simulink model "K_Sim_NoCap"  (R2020b)
settings: Solver=FixedStepAuto  StartTime=0  StopTime=2  FixedStep=Ts  RelTol=1e-3
undefined symbols (not defined in the file or in its folder): DeviceDiscreDamping, DevicePara, DevicePowerFlow, DeviceType, Fbase, OtherInputs, Sbase, Ts, Vbase, Wbase, x_e, Zbase
libraries: powerlib x155, SimplexPS x119
(part 1 of 2)
settings Model: Creator=admin_user  LastModifiedBy=admin_user

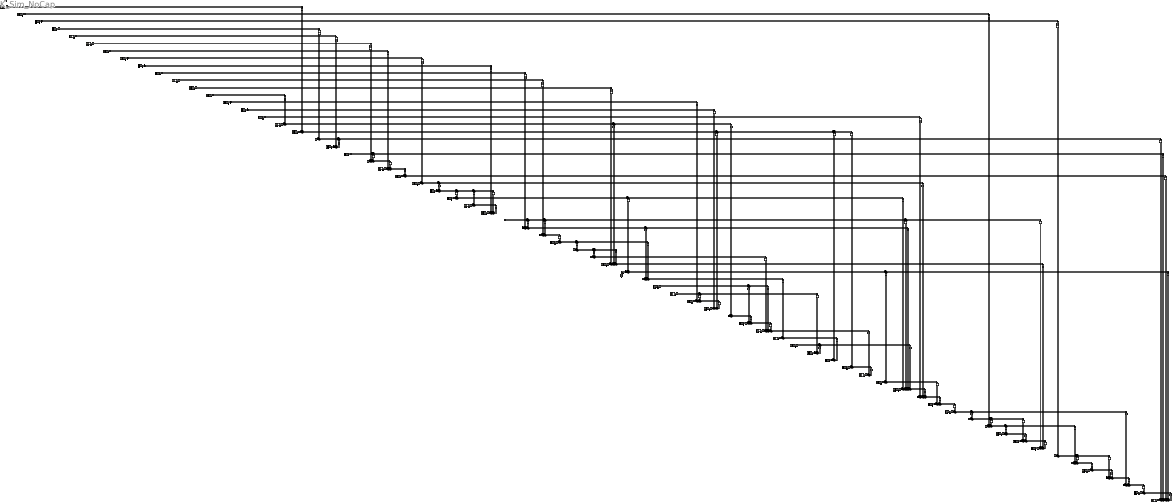
== system K_Sim_NoCap ==
  Branch1-18 : powerlib/Elements/Three-Phase Series RLC Branch  LConnTagsString=A|B|C  RConnTagsString=A|B|C  BranchType=RL  Resistance=(1e-07)*Zbase  Inductance=(0.003)*Zbase/Wbase  Capacitance=1e-6  Measurements=None
  Branch10-31 : powerlib/Elements/Three-Phase Series RLC Branch  LConnTagsString=A|B|C  RConnTagsString=A|B|C  BranchType=RL  Resistance=(1e-07)*Zbase  Inductance=(0.026)*Zbase/Wbase  Capacitance=1e-6  Measurements=None
  Branch11-32 : powerlib/Elements/Three-Phase Series RLC Branch  LConnTagsString=A|B|C  RConnTagsString=A|B|C  BranchType=RL  Resistance=(1e-07)*Zbase  Inductance=(0.013)*Zbase/Wbase  Capacitance=1e-6  Measurements=None
  Branch12-36 : powerlib/Elements/Three-Phase Series RLC Branch  LConnTagsString=A|B|C  RConnTagsString=A|B|C  BranchType=RL  Resistance=(1e-07)*Zbase  Inductance=(0.0075)*Zbase/Wbase  Capacitance=1e-6  Measurements=None
  Branch13-17 : powerlib/Elements/Three-Phase Series RLC Branch  LConnTagsString=A|B|C  RConnTagsString=A|B|C  BranchType=RL  Resistance=(1e-07)*Zbase  Inductance=(0.0033)*Zbase/Wbase  Capacitance=1e-6  Measurements=None
  Branch14-41 : powerlib/Elements/Three-Phase Series RLC Branch  LConnTagsString=A|B|C  RConnTagsString=A|B|C  BranchType=RL  Resistance=(1e-07)*Zbase  Inductance=(0.0015)*Zbase/Wbase  Capacitance=1e-6  Measurements=None
  Branch15-42 : powerlib/Elements/Three-Phase Series RLC Branch  LConnTagsString=A|B|C  RConnTagsString=A|B|C  BranchType=RL  Resistance=(1e-07)*Zbase  Inductance=(0.0015)*Zbase/Wbase  Capacitance=1e-6  Measurements=None
  Branch16-54 : powerlib/Elements/Three-Phase Series RLC Branch  LConnTagsString=A|B|C  RConnTagsString=A|B|C  BranchType=RL  Resistance=(1e-07)*Zbase  Inductance=(0.0181)*Zbase/Wbase  Capacitance=1e-6  Measurements=None
  Branch17-36 : powerlib/Elements/Three-Phase Series RLC Branch  LConnTagsString=A|B|C  RConnTagsString=A|B|C  BranchType=RL  Resistance=(0.0005)*Zbase  Inductance=(0.0045)*Zbase/Wbase  Capacitance=1e-6  Measurements=None
  Branch17-43 : powerlib/Elements/Three-Phase Series RLC Branch  LConnTagsString=A|B|C  RConnTagsString=A|B|C  BranchType=RL  Resistance=(0.0005)*Zbase  Inductance=(0.0276)*Zbase/Wbase  Capacitance=1e-6  Measurements=None
  Branch18-42 : powerlib/Elements/Three-Phase Series RLC Branch  LConnTagsString=A|B|C  RConnTagsString=A|B|C  BranchType=RL  Resistance=(0.004)*Zbase  Inductance=(0.06)*Zbase/Wbase  Capacitance=1e-6  Measurements=None
  Branch18-49 : powerlib/Elements/Three-Phase Series RLC Branch  LConnTagsString=A|B|C  RConnTagsString=A|B|C  BranchType=RL  Resistance=(0.0076)*Zbase  Inductance=(0.1141)*Zbase/Wbase  Capacitance=1e-6  Measurements=None
  Branch18-50 : powerlib/Elements/Three-Phase Series RLC Branch  LConnTagsString=A|B|C  RConnTagsString=A|B|C  BranchType=RL  Resistance=(0.0012)*Zbase  Inductance=(0.0288)*Zbase/Wbase  Capacitance=1e-6  Measurements=None
  Branch19-20 : powerlib/Elements/Three-Phase Series RLC Branch  LConnTagsString=A|B|C  RConnTagsString=A|B|C  BranchType=RL  Resistance=(0.00078652)*Zbase  Inductance=(0.015506)*Zbase/Wbase  Capacitance=1e-6  Measurements=None
  Branch19-68 : powerlib/Elements/Three-Phase Series RLC Branch  LConnTagsString=A|B|C  RConnTagsString=A|B|C  BranchType=RL  Resistance=(0.0016)*Zbase  Inductance=(0.0195)*Zbase/Wbase  Capacitance=1e-6  Measurements=None
  Branch2-58 : powerlib/Elements/Three-Phase Series RLC Branch  LConnTagsString=A|B|C  RConnTagsString=A|B|C  BranchType=RL  Resistance=(1e-07)*Zbase  Inductance=(0.025)*Zbase/Wbase  Capacitance=1e-6  Measurements=None
  Branch21-22 : powerlib/Elements/Three-Phase Series RLC Branch  LConnTagsString=A|B|C  RConnTagsString=A|B|C  BranchType=RL  Resistance=(0.0008)*Zbase  Inductance=(0.014)*Zbase/Wbase  Capacitance=1e-6  Measurements=None
  Branch21-68 : powerlib/Elements/Three-Phase Series RLC Branch  LConnTagsString=A|B|C  RConnTagsString=A|B|C  BranchType=RL  Resistance=(0.0008)*Zbase  Inductance=(0.0135)*Zbase/Wbase  Capacitance=1e-6  Measurements=None
  Branch22-23 : powerlib/Elements/Three-Phase Series RLC Branch  LConnTagsString=A|B|C  RConnTagsString=A|B|C  BranchType=RL  Resistance=(0.0006)*Zbase  Inductance=(0.0096)*Zbase/Wbase  Capacitance=1e-6  Measurements=None
  Branch23-24 : powerlib/Elements/Three-Phase Series RLC Branch  LConnTagsString=A|B|C  RConnTagsString=A|B|C  BranchType=RL  Resistance=(0.0022)*Zbase  Inductance=(0.035)*Zbase/Wbase  Capacitance=1e-6  Measurements=None
  Branch24-68 : powerlib/Elements/Three-Phase Series RLC Branch  LConnTagsString=A|B|C  RConnTagsString=A|B|C  BranchType=RL  Resistance=(0.0003)*Zbase  Inductance=(0.0059)*Zbase/Wbase  Capacitance=1e-6  Measurements=None
  Branch25-26 : powerlib/Elements/Three-Phase Series RLC Branch  LConnTagsString=A|B|C  RConnTagsString=A|B|C  BranchType=RL  Resistance=(0.0032)*Zbase  Inductance=(0.0323)*Zbase/Wbase  Capacitance=1e-6  Measurements=None
  Branch25-54 : powerlib/Elements/Three-Phase Series RLC Branch  LConnTagsString=A|B|C  RConnTagsString=A|B|C  BranchType=RL  Resistance=(0.007)*Zbase  Inductance=(0.0086)*Zbase/Wbase  Capacitance=1e-6  Measurements=None
  Branch26-27 : powerlib/Elements/Three-Phase Series RLC Branch  LConnTagsString=A|B|C  RConnTagsString=A|B|C  BranchType=RL  Resistance=(0.0014)*Zbase  Inductance=(0.0147)*Zbase/Wbase  Capacitance=1e-6  Measurements=None
  Branch26-28 : powerlib/Elements/Three-Phase Series RLC Branch  LConnTagsString=A|B|C  RConnTagsString=A|B|C  BranchType=RL  Resistance=(0.0043)*Zbase  Inductance=(0.0474)*Zbase/Wbase  Capacitance=1e-6  Measurements=None
  Branch26-29 : powerlib/Elements/Three-Phase Series RLC Branch  LConnTagsString=A|B|C  RConnTagsString=A|B|C  BranchType=RL  Resistance=(0.0057)*Zbase  Inductance=(0.0625)*Zbase/Wbase  Capacitance=1e-6  Measurements=None
  Branch27-37 : powerlib/Elements/Three-Phase Series RLC Branch  LConnTagsString=A|B|C  RConnTagsString=A|B|C  BranchType=RL  Resistance=(0.0013)*Zbase  Inductance=(0.0173)*Zbase/Wbase  Capacitance=1e-6  Measurements=None
  Branch27-53 : powerlib/Elements/Three-Phase Series RLC Branch  LConnTagsString=A|B|C  RConnTagsString=A|B|C  BranchType=RL  Resistance=(0.032)*Zbase  Inductance=(0.32)*Zbase/Wbase  Capacitance=1e-6  Measurements=None
  Branch28-29 : powerlib/Elements/Three-Phase Series RLC Branch  LConnTagsString=A|B|C  RConnTagsString=A|B|C  BranchType=RL  Resistance=(0.0014)*Zbase  Inductance=(0.0151)*Zbase/Wbase  Capacitance=1e-6  Measurements=None
  Branch3-62 : powerlib/Elements/Three-Phase Series RLC Branch  LConnTagsString=A|B|C  RConnTagsString=A|B|C  BranchType=RL  Resistance=(1e-07)*Zbase  Inductance=(0.02)*Zbase/Wbase  Capacitance=1e-6  Measurements=None
  Branch30-31 : powerlib/Elements/Three-Phase Series RLC Branch  LConnTagsString=A|B|C  RConnTagsString=A|B|C  BranchType=RL  Resistance=(0.0013)*Zbase  Inductance=(0.0187)*Zbase/Wbase  Capacitance=1e-6  Measurements=None
  Branch30-32 : powerlib/Elements/Three-Phase Series RLC Branch  LConnTagsString=A|B|C  RConnTagsString=A|B|C  BranchType=RL  Resistance=(0.0024)*Zbase  Inductance=(0.0288)*Zbase/Wbase  Capacitance=1e-6  Measurements=None
  Branch30-53 : powerlib/Elements/Three-Phase Series RLC Branch  LConnTagsString=A|B|C  RConnTagsString=A|B|C  BranchType=RL  Resistance=(0.0008)*Zbase  Inductance=(0.0074)*Zbase/Wbase  Capacitance=1e-6  Measurements=None
  Branch30-61 : powerlib/Elements/Three-Phase Series RLC Branch  LConnTagsString=A|B|C  RConnTagsString=A|B|C  BranchType=RL  Resistance=(0.00095)*Zbase  Inductance=(0.00915)*Zbase/Wbase  Capacitance=1e-6  Measurements=None
  Branch31-38 : powerlib/Elements/Three-Phase Series RLC Branch  LConnTagsString=A|B|C  RConnTagsString=A|B|C  BranchType=RL  Resistance=(0.0011)*Zbase  Inductance=(0.0147)*Zbase/Wbase  Capacitance=1e-6  Measurements=None
  Branch31-53 : powerlib/Elements/Three-Phase Series RLC Branch  LConnTagsString=A|B|C  RConnTagsString=A|B|C  BranchType=RL  Resistance=(0.0016)*Zbase  Inductance=(0.0163)*Zbase/Wbase  Capacitance=1e-6  Measurements=None
  Branch32-33 : powerlib/Elements/Three-Phase Series RLC Branch  LConnTagsString=A|B|C  RConnTagsString=A|B|C  BranchType=RL  Resistance=(0.0008)*Zbase  Inductance=(0.0099)*Zbase/Wbase  Capacitance=1e-6  Measurements=None
  Branch33-34 : powerlib/Elements/Three-Phase Series RLC Branch  LConnTagsString=A|B|C  RConnTagsString=A|B|C  BranchType=RL  Resistance=(0.0011)*Zbase  Inductance=(0.0157)*Zbase/Wbase  Capacitance=1e-6  Measurements=None
  Branch33-38 : powerlib/Elements/Three-Phase Series RLC Branch  LConnTagsString=A|B|C  RConnTagsString=A|B|C  BranchType=RL  Resistance=(0.0036)*Zbase  Inductance=(0.0444)*Zbase/Wbase  Capacitance=1e-6  Measurements=None
  Branch34-35 : powerlib/Elements/Three-Phase Series RLC Branch  LConnTagsString=A|B|C  RConnTagsString=A|B|C  BranchType=RL  Resistance=(0.0001)*Zbase  Inductance=(0.0074)*Zbase/Wbase  Capacitance=1e-6  Measurements=None
  Branch34-36 : powerlib/Elements/Three-Phase Series RLC Branch  LConnTagsString=A|B|C  RConnTagsString=A|B|C  BranchType=RL  Resistance=(0.0033)*Zbase  Inductance=(0.0111)*Zbase/Wbase  Capacitance=1e-6  Measurements=None
  Branch35-45 : powerlib/Elements/Three-Phase Series RLC Branch  LConnTagsString=A|B|C  RConnTagsString=A|B|C  BranchType=RL  Resistance=(0.0007)*Zbase  Inductance=(0.0175)*Zbase/Wbase  Capacitance=1e-6  Measurements=None
  Branch36-61 : powerlib/Elements/Three-Phase Series RLC Branch  LConnTagsString=A|B|C  RConnTagsString=A|B|C  BranchType=RL  Resistance=(0.0011)*Zbase  Inductance=(0.0098)*Zbase/Wbase  Capacitance=1e-6  Measurements=None
  Branch37-52 : powerlib/Elements/Three-Phase Series RLC Branch  LConnTagsString=A|B|C  RConnTagsString=A|B|C  BranchType=RL  Resistance=(0.0007)*Zbase  Inductance=(0.0082)*Zbase/Wbase  Capacitance=1e-6  Measurements=None
  Branch37-68 : powerlib/Elements/Three-Phase Series RLC Branch  LConnTagsString=A|B|C  RConnTagsString=A|B|C  BranchType=RL  Resistance=(0.0007)*Zbase  Inductance=(0.0089)*Zbase/Wbase  Capacitance=1e-6  Measurements=None
  Branch38-46 : powerlib/Elements/Three-Phase Series RLC Branch  LConnTagsString=A|B|C  RConnTagsString=A|B|C  BranchType=RL  Resistance=(0.0022)*Zbase  Inductance=(0.0284)*Zbase/Wbase  Capacitance=1e-6  Measurements=None
  Branch39-44 : powerlib/Elements/Three-Phase Series RLC Branch  LConnTagsString=A|B|C  RConnTagsString=A|B|C  BranchType=RL  Resistance=(1e-07)*Zbase  Inductance=(0.0411)*Zbase/Wbase  Capacitance=1e-6  Measurements=None
  Branch39-45 : powerlib/Elements/Three-Phase Series RLC Branch  LConnTagsString=A|B|C  RConnTagsString=A|B|C  BranchType=RL  Resistance=(1e-07)*Zbase  Inductance=(0.0839)*Zbase/Wbase  Capacitance=1e-6  Measurements=None
  Branch4-19 : powerlib/Elements/Three-Phase Series RLC Branch  LConnTagsString=A|B|C  RConnTagsString=A|B|C  BranchType=RL  Resistance=(0.0007)*Zbase  Inductance=(0.0142)*Zbase/Wbase  Capacitance=1e-6  Measurements=None
  Branch40-41 : powerlib/Elements/Three-Phase Series RLC Branch  LConnTagsString=A|B|C  RConnTagsString=A|B|C  BranchType=RL  Resistance=(0.006)*Zbase  Inductance=(0.084)*Zbase/Wbase  Capacitance=1e-6  Measurements=None
  Branch40-48 : powerlib/Elements/Three-Phase Series RLC Branch  LConnTagsString=A|B|C  RConnTagsString=A|B|C  BranchType=RL  Resistance=(0.002)*Zbase  Inductance=(0.022)*Zbase/Wbase  Capacitance=1e-6  Measurements=None
  Branch41-42 : powerlib/Elements/Three-Phase Series RLC Branch  LConnTagsString=A|B|C  RConnTagsString=A|B|C  BranchType=RL  Resistance=(0.004)*Zbase  Inductance=(0.06)*Zbase/Wbase  Capacitance=1e-6  Measurements=None
  Branch43-44 : powerlib/Elements/Three-Phase Series RLC Branch  LConnTagsString=A|B|C  RConnTagsString=A|B|C  BranchType=RL  Resistance=(0.0001)*Zbase  Inductance=(0.0011)*Zbase/Wbase  Capacitance=1e-6  Measurements=None
  Branch44-45 : powerlib/Elements/Three-Phase Series RLC Branch  LConnTagsString=A|B|C  RConnTagsString=A|B|C  BranchType=RL  Resistance=(0.0025)*Zbase  Inductance=(0.073)*Zbase/Wbase  Capacitance=1e-6  Measurements=None
  Branch45-51 : powerlib/Elements/Three-Phase Series RLC Branch  LConnTagsString=A|B|C  RConnTagsString=A|B|C  BranchType=RL  Resistance=(0.0004)*Zbase  Inductance=(0.0105)*Zbase/Wbase  Capacitance=1e-6  Measurements=None
  Branch46-49 : powerlib/Elements/Three-Phase Series RLC Branch  LConnTagsString=A|B|C  RConnTagsString=A|B|C  BranchType=RL  Resistance=(0.0018)*Zbase  Inductance=(0.0274)*Zbase/Wbase  Capacitance=1e-6  Measurements=None
  Branch47-48 : powerlib/Elements/Three-Phase Series RLC Branch  LConnTagsString=A|B|C  RConnTagsString=A|B|C  BranchType=RL  Resistance=(0.00125)*Zbase  Inductance=(0.0134)*Zbase/Wbase  Capacitance=1e-6  Measurements=None
  Branch47-53 : powerlib/Elements/Three-Phase Series RLC Branch  LConnTagsString=A|B|C  RConnTagsString=A|B|C  BranchType=RL  Resistance=(0.0013)*Zbase  Inductance=(0.0188)*Zbase/Wbase  Capacitance=1e-6  Measurements=None
  Branch5-20 : powerlib/Elements/Three-Phase Series RLC Branch  LConnTagsString=A|B|C  RConnTagsString=A|B|C  BranchType=RL  Resistance=(0.0009)*Zbase  Inductance=(0.018)*Zbase/Wbase  Capacitance=1e-6  Measurements=None
  Branch50-51 : powerlib/Elements/Three-Phase Series RLC Branch  LConnTagsString=A|B|C  RConnTagsString=A|B|C  BranchType=RL  Resistance=(0.0009)*Zbase  Inductance=(0.0221)*Zbase/Wbase  Capacitance=1e-6  Measurements=None
  Branch52-55 : powerlib/Elements/Three-Phase Series RLC Branch  LConnTagsString=A|B|C  RConnTagsString=A|B|C  BranchType=RL  Resistance=(0.0011)*Zbase  Inductance=(0.0133)*Zbase/Wbase  Capacitance=1e-6  Measurements=None
  Branch53-54 : powerlib/Elements/Three-Phase Series RLC Branch  LConnTagsString=A|B|C  RConnTagsString=A|B|C  BranchType=RL  Resistance=(0.0035)*Zbase  Inductance=(0.0411)*Zbase/Wbase  Capacitance=1e-6  Measurements=None
  Branch54-55 : powerlib/Elements/Three-Phase Series RLC Branch  LConnTagsString=A|B|C  RConnTagsString=A|B|C  BranchType=RL  Resistance=(0.0013)*Zbase  Inductance=(0.0151)*Zbase/Wbase  Capacitance=1e-6  Measurements=None
  Branch55-56 : powerlib/Elements/Three-Phase Series RLC Branch  LConnTagsString=A|B|C  RConnTagsString=A|B|C  BranchType=RL  Resistance=(0.0013)*Zbase  Inductance=(0.0213)*Zbase/Wbase  Capacitance=1e-6  Measurements=None
  Branch56-57 : powerlib/Elements/Three-Phase Series RLC Branch  LConnTagsString=A|B|C  RConnTagsString=A|B|C  BranchType=RL  Resistance=(0.0008)*Zbase  Inductance=(0.0128)*Zbase/Wbase  Capacitance=1e-6  Measurements=None
  Branch56-66 : powerlib/Elements/Three-Phase Series RLC Branch  LConnTagsString=A|B|C  RConnTagsString=A|B|C  BranchType=RL  Resistance=(0.0008)*Zbase  Inductance=(0.0129)*Zbase/Wbase  Capacitance=1e-6  Measurements=None
  Branch57-58 : powerlib/Elements/Three-Phase Series RLC Branch  LConnTagsString=A|B|C  RConnTagsString=A|B|C  BranchType=RL  Resistance=(0.0002)*Zbase  Inductance=(0.0026)*Zbase/Wbase  Capacitance=1e-6  Measurements=None
  Branch57-60 : powerlib/Elements/Three-Phase Series RLC Branch  LConnTagsString=A|B|C  RConnTagsString=A|B|C  BranchType=RL  Resistance=(0.0008)*Zbase  Inductance=(0.0112)*Zbase/Wbase  Capacitance=1e-6  Measurements=None
  Branch58-59 : powerlib/Elements/Three-Phase Series RLC Branch  LConnTagsString=A|B|C  RConnTagsString=A|B|C  BranchType=RL  Resistance=(0.0006)*Zbase  Inductance=(0.0092)*Zbase/Wbase  Capacitance=1e-6  Measurements=None
  Branch58-63 : powerlib/Elements/Three-Phase Series RLC Branch  LConnTagsString=A|B|C  RConnTagsString=A|B|C  BranchType=RL  Resistance=(0.0007)*Zbase  Inductance=(0.0082)*Zbase/Wbase  Capacitance=1e-6  Measurements=None
  Branch59-60 : powerlib/Elements/Three-Phase Series RLC Branch  LConnTagsString=A|B|C  RConnTagsString=A|B|C  BranchType=RL  Resistance=(0.0004)*Zbase  Inductance=(0.0046)*Zbase/Wbase  Capacitance=1e-6  Measurements=None
  Branch6-22 : powerlib/Elements/Three-Phase Series RLC Branch  LConnTagsString=A|B|C  RConnTagsString=A|B|C  BranchType=RL  Resistance=(1e-07)*Zbase  Inductance=(0.0143)*Zbase/Wbase  Capacitance=1e-6  Measurements=None
  Branch60-61 : powerlib/Elements/Three-Phase Series RLC Branch  LConnTagsString=A|B|C  RConnTagsString=A|B|C  BranchType=RL  Resistance=(0.0023)*Zbase  Inductance=(0.0363)*Zbase/Wbase  Capacitance=1e-6  Measurements=None
  Branch62-63 : powerlib/Elements/Three-Phase Series RLC Branch  LConnTagsString=A|B|C  RConnTagsString=A|B|C  BranchType=RL  Resistance=(0.0004)*Zbase  Inductance=(0.0043)*Zbase/Wbase  Capacitance=1e-6  Measurements=None
  Branch62-65 : powerlib/Elements/Three-Phase Series RLC Branch  LConnTagsString=A|B|C  RConnTagsString=A|B|C  BranchType=RL  Resistance=(0.0004)*Zbase  Inductance=(0.0043)*Zbase/Wbase  Capacitance=1e-6  Measurements=None
  Branch63-64 : powerlib/Elements/Three-Phase Series RLC Branch  LConnTagsString=A|B|C  RConnTagsString=A|B|C  BranchType=RL  Resistance=(0.0016)*Zbase  Inductance=(0.0435)*Zbase/Wbase  Capacitance=1e-6  Measurements=None
  Branch64-65 : powerlib/Elements/Three-Phase Series RLC Branch  LConnTagsString=A|B|C  RConnTagsString=A|B|C  BranchType=RL  Resistance=(0.0017978)*Zbase  Inductance=(0.048877)*Zbase/Wbase  Capacitance=1e-6  Measurements=None
  Branch65-66 : powerlib/Elements/Three-Phase Series RLC Branch  LConnTagsString=A|B|C  RConnTagsString=A|B|C  BranchType=RL  Resistance=(0.0009)*Zbase  Inductance=(0.0101)*Zbase/Wbase  Capacitance=1e-6  Measurements=None
  Branch66-67 : powerlib/Elements/Three-Phase Series RLC Branch  LConnTagsString=A|B|C  RConnTagsString=A|B|C  BranchType=RL  Resistance=(0.0018)*Zbase  Inductance=(0.0217)*Zbase/Wbase  Capacitance=1e-6  Measurements=None
  Branch67-68 : powerlib/Elements/Three-Phase Series RLC Branch  LConnTagsString=A|B|C  RConnTagsString=A|B|C  BranchType=RL  Resistance=(0.0009)*Zbase  Inductance=(0.0094)*Zbase/Wbase  Capacitance=1e-6  Measurements=None
  Branch7-23 : powerlib/Elements/Three-Phase Series RLC Branch  LConnTagsString=A|B|C  RConnTagsString=A|B|C  BranchType=RL  Resistance=(0.0005)*Zbase  Inductance=(0.0272)*Zbase/Wbase  Capacitance=1e-6  Measurements=None
  Branch8-25 : powerlib/Elements/Three-Phase Series RLC Branch  LConnTagsString=A|B|C  RConnTagsString=A|B|C  BranchType=RL  Resistance=(0.0006)*Zbase  Inductance=(0.0232)*Zbase/Wbase  Capacitance=1e-6  Measurements=None
  Branch9-29 : powerlib/Elements/Three-Phase Series RLC Branch  LConnTagsString=A|B|C  RConnTagsString=A|B|C  BranchType=RL  Resistance=(0.0008)*Zbase  Inductance=(0.0156)*Zbase/Wbase  Capacitance=1e-6  Measurements=None
  Bus{1..68} (68 alike) : SimplexPS/Three-Phase Bus  Vbase=1  Sbase=1
      settings: SourceProductName=Simplex Power Systems
  Current Measurement1 : powerlib/Measurements/Current Measurement  PhasorSimulation=off  OutputType=Complex  PSBequivalent=0
  D-GND{1..18,20..29,33,36,39..42,44..53,55..56,59..61,64,67..68} (52 alike) : powerlib/Elements/Ground  LConnTagsString=a
  D-Scope{1..18,20..21,23..29,33,36,39..42,44..53,55..56,59..61,64,67..68} (51 alike) : Scope  NumInputPorts=7
  DS-Bus{1..18,20..21,23..29,33,36,39..42,44..53,55..56,59..61,64,67..68} (51 alike) : BusSelector  OutputSignals=v_dq,i_dq,v_abc,i_abc,w,theta,pq
  Load Impulse1 : Subsystem  AncestorBlock=SimplexPS/Load Impulse  mask{t0=1, dt=3/60, R=1e-9*Zbase}
  Scope1 : Scope
  Transformer10-31 : powerlib/Elements/Three-Phase Transformer (Two Windings)  Winding1Connection=Yg  Winding2Connection=Yg  CoreType=Three single-phase transformers  SetSaturation=off  Hysteresis=off  DataFile='hysteresis'  SetInitialFlux=off  Measurements=None  UNITS=pu  NominalPower=[Sbase, Fbase]  Winding1=[1.04*Vbase, 0, 0]  Winding2=[Vbase, 0, 0]  Rm=1e4  Lm=1e4  L0=0.5  Saturation=[ 0,0 ; 0.0024,1.2 ; 1.0,1.52 ]  InitialFluxes=[ 0.8 , -0.8 , 0.7 ]  BreakLoop=off  DiscreteSolver=Trapezoidal iterative  DataType=off  TransfoNumber=1
  Transformer11-32 : powerlib/Elements/Three-Phase Transformer (Two Windings)  Winding1Connection=Yg  Winding2Connection=Yg  CoreType=Three single-phase transformers  SetSaturation=off  Hysteresis=off  DataFile='hysteresis'  SetInitialFlux=off  Measurements=None  UNITS=pu  NominalPower=[Sbase, Fbase]  Winding1=[1.04*Vbase, 0, 0]  Winding2=[Vbase, 0, 0]  Rm=1e4  Lm=1e4  L0=0.5  Saturation=[ 0,0 ; 0.0024,1.2 ; 1.0,1.52 ]  InitialFluxes=[ 0.8 , -0.8 , 0.7 ]  BreakLoop=off  DiscreteSolver=Trapezoidal iterative  DataType=off  TransfoNumber=1
  Transformer12-36 : powerlib/Elements/Three-Phase Transformer (Two Windings)  Winding1Connection=Yg  Winding2Connection=Yg  CoreType=Three single-phase transformers  SetSaturation=off  Hysteresis=off  DataFile='hysteresis'  SetInitialFlux=off  Measurements=None  UNITS=pu  NominalPower=[Sbase, Fbase]  Winding1=[1.04*Vbase, 0, 0]  Winding2=[Vbase, 0, 0]  Rm=1e4  Lm=1e4  L0=0.5  Saturation=[ 0,0 ; 0.0024,1.2 ; 1.0,1.52 ]  InitialFluxes=[ 0.8 , -0.8 , 0.7 ]  BreakLoop=off  DiscreteSolver=Trapezoidal iterative  DataType=off  TransfoNumber=1
  Transformer13-17 : powerlib/Elements/Three-Phase Transformer (Two Windings)  Winding1Connection=Yg  Winding2Connection=Yg  CoreType=Three single-phase transformers  SetSaturation=off  Hysteresis=off  DataFile='hysteresis'  SetInitialFlux=off  Measurements=None  UNITS=pu  NominalPower=[Sbase, Fbase]  Winding1=[1.04*Vbase, 0, 0]  Winding2=[Vbase, 0, 0]  Rm=1e4  Lm=1e4  L0=0.5  Saturation=[ 0,0 ; 0.0024,1.2 ; 1.0,1.52 ]  InitialFluxes=[ 0.8 , -0.8 , 0.7 ]  BreakLoop=off  DiscreteSolver=Trapezoidal iterative  DataType=off  TransfoNumber=1
  Transformer16-54 : powerlib/Elements/Three-Phase Transformer (Two Windings)  Winding1Connection=Yg  Winding2Connection=Yg  CoreType=Three single-phase transformers  SetSaturation=off  Hysteresis=off  DataFile='hysteresis'  SetInitialFlux=off  Measurements=None  UNITS=pu  NominalPower=[Sbase, Fbase]  Winding1=[1.025*Vbase, 0, 0]  Winding2=[Vbase, 0, 0]  Rm=1e4  Lm=1e4  L0=0.5  Saturation=[ 0,0 ; 0.0024,1.2 ; 1.0,1.52 ]  InitialFluxes=[ 0.8 , -0.8 , 0.7 ]  BreakLoop=off  DiscreteSolver=Trapezoidal iterative  DataType=off  TransfoNumber=1
  Transformer19-20 : powerlib/Elements/Three-Phase Transformer (Two Windings)  Winding1Connection=Yg  Winding2Connection=Yg  CoreType=Three single-phase transformers  SetSaturation=off  Hysteresis=off  DataFile='hysteresis'  SetInitialFlux=off  Measurements=None  UNITS=pu  NominalPower=[Sbase, Fbase]  Winding1=[0.9434*Vbase, 0, 0]  Winding2=[Vbase, 0, 0]  Rm=1e4  Lm=1e4  L0=0.5  Saturation=[ 0,0 ; 0.0024,1.2 ; 1.0,1.52 ]  InitialFluxes=[ 0.8 , -0.8 , 0.7 ]  BreakLoop=off  DiscreteSolver=Trapezoidal iterative  DataType=off  TransfoNumber=1
  Transformer2-58 : powerlib/Elements/Three-Phase Transformer (Two Windings)  Winding1Connection=Yg  Winding2Connection=Yg  CoreType=Three single-phase transformers  SetSaturation=off  Hysteresis=off  DataFile='hysteresis'  SetInitialFlux=off  Measurements=None  UNITS=pu  NominalPower=[Sbase, Fbase]  Winding1=[1.07*Vbase, 0, 0]  Winding2=[Vbase, 0, 0]  Rm=1e4  Lm=1e4  L0=0.5  Saturation=[ 0,0 ; 0.0024,1.2 ; 1.0,1.52 ]  InitialFluxes=[ 0.8 , -0.8 , 0.7 ]  BreakLoop=off  DiscreteSolver=Trapezoidal iterative  DataType=off  TransfoNumber=1
  Transformer3-62 : powerlib/Elements/Three-Phase Transformer (Two Windings)  Winding1Connection=Yg  Winding2Connection=Yg  CoreType=Three single-phase transformers  SetSaturation=off  Hysteresis=off  DataFile='hysteresis'  SetInitialFlux=off  Measurements=None  UNITS=pu  NominalPower=[Sbase, Fbase]  Winding1=[1.07*Vbase, 0, 0]  Winding2=[Vbase, 0, 0]  Rm=1e4  Lm=1e4  L0=0.5  Saturation=[ 0,0 ; 0.0024,1.2 ; 1.0,1.52 ]  InitialFluxes=[ 0.8 , -0.8 , 0.7 ]  BreakLoop=off  DiscreteSolver=Trapezoidal iterative  DataType=off  TransfoNumber=1
  Transformer34-35 : powerlib/Elements/Three-Phase Transformer (Two Windings)  Winding1Connection=Yg  Winding2Connection=Yg  CoreType=Three single-phase transformers  SetSaturation=off  Hysteresis=off  DataFile='hysteresis'  SetInitialFlux=off  Measurements=None  UNITS=pu  NominalPower=[Sbase, Fbase]  Winding1=[0.946*Vbase, 0, 0]  Winding2=[Vbase, 0, 0]  Rm=1e4  Lm=1e4  L0=0.5  Saturation=[ 0,0 ; 0.0024,1.2 ; 1.0,1.52 ]  InitialFluxes=[ 0.8 , -0.8 , 0.7 ]  BreakLoop=off  DiscreteSolver=Trapezoidal iterative  DataType=off  TransfoNumber=1
  Transformer4-19 : powerlib/Elements/Three-Phase Transformer (Two Windings)  Winding1Connection=Yg  Winding2Connection=Yg  CoreType=Three single-phase transformers  SetSaturation=off  Hysteresis=off  DataFile='hysteresis'  SetInitialFlux=off  Measurements=None  UNITS=pu  NominalPower=[Sbase, Fbase]  Winding1=[1.07*Vbase, 0, 0]  Winding2=[Vbase, 0, 0]  Rm=1e4  Lm=1e4  L0=0.5  Saturation=[ 0,0 ; 0.0024,1.2 ; 1.0,1.52 ]  InitialFluxes=[ 0.8 , -0.8 , 0.7 ]  BreakLoop=off  DiscreteSolver=Trapezoidal iterative  DataType=off  TransfoNumber=1
  Transformer5-20 : powerlib/Elements/Three-Phase Transformer (Two Windings)  Winding1Connection=Yg  Winding2Connection=Yg  CoreType=Three single-phase transformers  SetSaturation=off  Hysteresis=off  DataFile='hysteresis'  SetInitialFlux=off  Measurements=None  UNITS=pu  NominalPower=[Sbase, Fbase]  Winding1=[1.009*Vbase, 0, 0]  Winding2=[Vbase, 0, 0]  Rm=1e4  Lm=1e4  L0=0.5  Saturation=[ 0,0 ; 0.0024,1.2 ; 1.0,1.52 ]  InitialFluxes=[ 0.8 , -0.8 , 0.7 ]  BreakLoop=off  DiscreteSolver=Trapezoidal iterative  DataType=off  TransfoNumber=1
  Transformer6-22 : powerlib/Elements/Three-Phase Transformer (Two Windings)  Winding1Connection=Yg  Winding2Connection=Yg  CoreType=Three single-phase transformers  SetSaturation=off  Hysteresis=off  DataFile='hysteresis'  SetInitialFlux=off  Measurements=None  UNITS=pu  NominalPower=[Sbase, Fbase]  Winding1=[1.025*Vbase, 0, 0]  Winding2=[Vbase, 0, 0]  Rm=1e4  Lm=1e4  L0=0.5  Saturation=[ 0,0 ; 0.0024,1.2 ; 1.0,1.52 ]  InitialFluxes=[ 0.8 , -0.8 , 0.7 ]  BreakLoop=off  DiscreteSolver=Trapezoidal iterative  DataType=off  TransfoNumber=1
  Transformer63-64 : powerlib/Elements/Three-Phase Transformer (Two Windings)  Winding1Connection=Yg  Winding2Connection=Yg  CoreType=Three single-phase transformers  SetSaturation=off  Hysteresis=off  DataFile='hysteresis'  SetInitialFlux=off  Measurements=None  UNITS=pu  NominalPower=[Sbase, Fbase]  Winding1=[1.06*Vbase, 0, 0]  Winding2=[Vbase, 0, 0]  Rm=1e4  Lm=1e4  L0=0.5  Saturation=[ 0,0 ; 0.0024,1.2 ; 1.0,1.52 ]  InitialFluxes=[ 0.8 , -0.8 , 0.7 ]  BreakLoop=off  DiscreteSolver=Trapezoidal iterative  DataType=off  TransfoNumber=1
  Transformer64-65 : powerlib/Elements/Three-Phase Transformer (Two Windings)  Winding1Connection=Yg  Winding2Connection=Yg  CoreType=Three single-phase transformers  SetSaturation=off  Hysteresis=off  DataFile='hysteresis'  SetInitialFlux=off  Measurements=None  UNITS=pu  NominalPower=[Sbase, Fbase]  Winding1=[0.9434*Vbase, 0, 0]  Winding2=[Vbase, 0, 0]  Rm=1e4  Lm=1e4  L0=0.5  Saturation=[ 0,0 ; 0.0024,1.2 ; 1.0,1.52 ]  InitialFluxes=[ 0.8 , -0.8 , 0.7 ]  BreakLoop=off  DiscreteSolver=Trapezoidal iterative  DataType=off  TransfoNumber=1
  Transformer8-25 : powerlib/Elements/Three-Phase Transformer (Two Windings)  Winding1Connection=Yg  Winding2Connection=Yg  CoreType=Three single-phase transformers  SetSaturation=off  Hysteresis=off  DataFile='hysteresis'  SetInitialFlux=off  Measurements=None  UNITS=pu  NominalPower=[Sbase, Fbase]  Winding1=[1.025*Vbase, 0, 0]  Winding2=[Vbase, 0, 0]  Rm=1e4  Lm=1e4  L0=0.5  Saturation=[ 0,0 ; 0.0024,1.2 ; 1.0,1.52 ]  InitialFluxes=[ 0.8 , -0.8 , 0.7 ]  BreakLoop=off  DiscreteSolver=Trapezoidal iterative  DataType=off  TransfoNumber=1
  Transformer9-29 : powerlib/Elements/Three-Phase Transformer (Two Windings)  Winding1Connection=Yg  Winding2Connection=Yg  CoreType=Three single-phase transformers  SetSaturation=off  Hysteresis=off  DataFile='hysteresis'  SetInitialFlux=off  Measurements=None  UNITS=pu  NominalPower=[Sbase, Fbase]  Winding1=[1.025*Vbase, 0, 0]  Winding2=[Vbase, 0, 0]  Rm=1e4  Lm=1e4  L0=0.5  Saturation=[ 0,0 ; 0.0024,1.2 ; 1.0,1.52 ]  InitialFluxes=[ 0.8 , -0.8 , 0.7 ]  BreakLoop=off  DiscreteSolver=Trapezoidal iterative  DataType=off  TransfoNumber=1
  VSI-PLL1 : SimplexPS/Grid-Following Voltage-Source Inverter (dq-Frame System Object)  Ts=Ts  Sbase=Sbase  Vbase=Vbase  Wbase=Wbase  DeviceType=DeviceType{1}  DevicePara=DevicePara{1}  PowerFlow=DevicePowerFlow{1}  x0=x_e{1}  OtherInputs=OtherInputs{1}  DiscreMethod=Hybrid Trapezoidal  EnableInsideModification=off  DiscreDampingFlag=on  DiscreDampingValue=DeviceDiscreDamping{1}  LinearizationTimes=1  DirectFeedthrough=off
      settings: SourceProductName=Simplex Power Systems
  VSI-PLL10 : SimplexPS/Grid-Following Voltage-Source Inverter (dq-Frame System Object)  Ts=Ts  Sbase=Sbase  Vbase=Vbase  Wbase=Wbase  DeviceType=DeviceType{10}  DevicePara=DevicePara{10}  PowerFlow=DevicePowerFlow{10}  x0=x_e{10}  OtherInputs=OtherInputs{10}  DiscreMethod=Hybrid Trapezoidal  EnableInsideModification=off  DiscreDampingFlag=on  DiscreDampingValue=DeviceDiscreDamping{10}  LinearizationTimes=1  DirectFeedthrough=off
      settings: SourceProductName=Simplex Power Systems
  VSI-PLL11 : SimplexPS/Grid-Following Voltage-Source Inverter (dq-Frame System Object)  Ts=Ts  Sbase=Sbase  Vbase=Vbase  Wbase=Wbase  DeviceType=DeviceType{11}  DevicePara=DevicePara{11}  PowerFlow=DevicePowerFlow{11}  x0=x_e{11}  OtherInputs=OtherInputs{11}  DiscreMethod=Hybrid Trapezoidal  EnableInsideModification=off  DiscreDampingFlag=on  DiscreDampingValue=DeviceDiscreDamping{11}  LinearizationTimes=1  DirectFeedthrough=off
      settings: SourceProductName=Simplex Power Systems
  VSI-PLL12 : SimplexPS/Grid-Following Voltage-Source Inverter (dq-Frame System Object)  Ts=Ts  Sbase=Sbase  Vbase=Vbase  Wbase=Wbase  DeviceType=DeviceType{12}  DevicePara=DevicePara{12}  PowerFlow=DevicePowerFlow{12}  x0=x_e{12}  OtherInputs=OtherInputs{12}  DiscreMethod=Hybrid Trapezoidal  EnableInsideModification=off  DiscreDampingFlag=on  DiscreDampingValue=DeviceDiscreDamping{12}  LinearizationTimes=1  DirectFeedthrough=off
      settings: SourceProductName=Simplex Power Systems
  VSI-PLL13 : SimplexPS/Grid-Following Voltage-Source Inverter (dq-Frame System Object)  Ts=Ts  Sbase=Sbase  Vbase=Vbase  Wbase=Wbase  DeviceType=DeviceType{13}  DevicePara=DevicePara{13}  PowerFlow=DevicePowerFlow{13}  x0=x_e{13}  OtherInputs=OtherInputs{13}  DiscreMethod=Hybrid Trapezoidal  EnableInsideModification=off  DiscreDampingFlag=on  DiscreDampingValue=DeviceDiscreDamping{13}  LinearizationTimes=1  DirectFeedthrough=off
      settings: SourceProductName=Simplex Power Systems
  VSI-PLL14 : SimplexPS/Grid-Following Voltage-Source Inverter (dq-Frame System Object)  Ts=Ts  Sbase=Sbase  Vbase=Vbase  Wbase=Wbase  DeviceType=DeviceType{14}  DevicePara=DevicePara{14}  PowerFlow=DevicePowerFlow{14}  x0=x_e{14}  OtherInputs=OtherInputs{14}  DiscreMethod=Hybrid Trapezoidal  EnableInsideModification=off  DiscreDampingFlag=on  DiscreDampingValue=DeviceDiscreDamping{14}  LinearizationTimes=1  DirectFeedthrough=off
      settings: SourceProductName=Simplex Power Systems
  VSI-PLL15 : SimplexPS/Grid-Following Voltage-Source Inverter (dq-Frame System Object)  Ts=Ts  Sbase=Sbase  Vbase=Vbase  Wbase=Wbase  DeviceType=DeviceType{15}  DevicePara=DevicePara{15}  PowerFlow=DevicePowerFlow{15}  x0=x_e{15}  OtherInputs=OtherInputs{15}  DiscreMethod=Hybrid Trapezoidal  EnableInsideModification=off  DiscreDampingFlag=on  DiscreDampingValue=DeviceDiscreDamping{15}  LinearizationTimes=1  DirectFeedthrough=off
      settings: SourceProductName=Simplex Power Systems
  VSI-PLL16 : SimplexPS/Grid-Following Voltage-Source Inverter (dq-Frame System Object)  Ts=Ts  Sbase=Sbase  Vbase=Vbase  Wbase=Wbase  DeviceType=DeviceType{16}  DevicePara=DevicePara{16}  PowerFlow=DevicePowerFlow{16}  x0=x_e{16}  OtherInputs=OtherInputs{16}  DiscreMethod=Hybrid Trapezoidal  EnableInsideModification=off  DiscreDampingFlag=on  DiscreDampingValue=DeviceDiscreDamping{16}  LinearizationTimes=1  DirectFeedthrough=off
      settings: SourceProductName=Simplex Power Systems
  VSI-PLL17 : SimplexPS/Grid-Following Voltage-Source Inverter (dq-Frame System Object)  Ts=Ts  Sbase=Sbase  Vbase=Vbase  Wbase=Wbase  DeviceType=DeviceType{17}  DevicePara=DevicePara{17}  PowerFlow=DevicePowerFlow{17}  x0=x_e{17}  OtherInputs=OtherInputs{17}  DiscreMethod=Hybrid Trapezoidal  EnableInsideModification=off  DiscreDampingFlag=on  DiscreDampingValue=DeviceDiscreDamping{17}  LinearizationTimes=1  DirectFeedthrough=off
      settings: SourceProductName=Simplex Power Systems
  VSI-PLL18 : SimplexPS/Grid-Following Voltage-Source Inverter (dq-Frame System Object)  Ts=Ts  Sbase=Sbase  Vbase=Vbase  Wbase=Wbase  DeviceType=DeviceType{18}  DevicePara=DevicePara{18}  PowerFlow=DevicePowerFlow{18}  x0=x_e{18}  OtherInputs=OtherInputs{18}  DiscreMethod=Hybrid Trapezoidal  EnableInsideModification=off  DiscreDampingFlag=on  DiscreDampingValue=DeviceDiscreDamping{18}  LinearizationTimes=1  DirectFeedthrough=off
      settings: SourceProductName=Simplex Power Systems
  VSI-PLL2 : SimplexPS/Grid-Following Voltage-Source Inverter (dq-Frame System Object)  Ts=Ts  Sbase=Sbase  Vbase=Vbase  Wbase=Wbase  DeviceType=DeviceType{2}  DevicePara=DevicePara{2}  PowerFlow=DevicePowerFlow{2}  x0=x_e{2}  OtherInputs=OtherInputs{2}  DiscreMethod=Hybrid Trapezoidal  EnableInsideModification=off  DiscreDampingFlag=on  DiscreDampingValue=DeviceDiscreDamping{2}  LinearizationTimes=1  DirectFeedthrough=off
      settings: SourceProductName=Simplex Power Systems
  VSI-PLL20 : SimplexPS/Grid-Following Voltage-Source Inverter (dq-Frame System Object)  Ts=Ts  Sbase=Sbase  Vbase=Vbase  Wbase=Wbase  DeviceType=DeviceType{20}  DevicePara=DevicePara{20}  PowerFlow=DevicePowerFlow{20}  x0=x_e{20}  OtherInputs=OtherInputs{20}  DiscreMethod=Hybrid Trapezoidal  EnableInsideModification=off  DiscreDampingFlag=on  DiscreDampingValue=DeviceDiscreDamping{20}  LinearizationTimes=1  DirectFeedthrough=off
      settings: SourceProductName=Simplex Power Systems
  VSI-PLL21 : SimplexPS/Grid-Following Voltage-Source Inverter (dq-Frame System Object)  Ts=Ts  Sbase=Sbase  Vbase=Vbase  Wbase=Wbase  DeviceType=DeviceType{21}  DevicePara=DevicePara{21}  PowerFlow=DevicePowerFlow{21}  x0=x_e{21}  OtherInputs=OtherInputs{21}  DiscreMethod=Hybrid Trapezoidal  EnableInsideModification=off  DiscreDampingFlag=on  DiscreDampingValue=DeviceDiscreDamping{21}  LinearizationTimes=1  DirectFeedthrough=off
      settings: SourceProductName=Simplex Power Systems
  VSI-PLL23 : SimplexPS/Grid-Following Voltage-Source Inverter (dq-Frame System Object)  Ts=Ts  Sbase=Sbase  Vbase=Vbase  Wbase=Wbase  DeviceType=DeviceType{23}  DevicePara=DevicePara{23}  PowerFlow=DevicePowerFlow{23}  x0=x_e{23}  OtherInputs=OtherInputs{23}  DiscreMethod=Hybrid Trapezoidal  EnableInsideModification=off  DiscreDampingFlag=on  DiscreDampingValue=DeviceDiscreDamping{23}  LinearizationTimes=1  DirectFeedthrough=off
      settings: SourceProductName=Simplex Power Systems
  VSI-PLL24 : SimplexPS/Grid-Following Voltage-Source Inverter (dq-Frame System Object)  Ts=Ts  Sbase=Sbase  Vbase=Vbase  Wbase=Wbase  DeviceType=DeviceType{24}  DevicePara=DevicePara{24}  PowerFlow=DevicePowerFlow{24}  x0=x_e{24}  OtherInputs=OtherInputs{24}  DiscreMethod=Hybrid Trapezoidal  EnableInsideModification=off  DiscreDampingFlag=on  DiscreDampingValue=DeviceDiscreDamping{24}  LinearizationTimes=1  DirectFeedthrough=off
      settings: SourceProductName=Simplex Power Systems
  VSI-PLL25 : SimplexPS/Grid-Following Voltage-Source Inverter (dq-Frame System Object)  Ts=Ts  Sbase=Sbase  Vbase=Vbase  Wbase=Wbase  DeviceType=DeviceType{25}  DevicePara=DevicePara{25}  PowerFlow=DevicePowerFlow{25}  x0=x_e{25}  OtherInputs=OtherInputs{25}  DiscreMethod=Hybrid Trapezoidal  EnableInsideModification=off  DiscreDampingFlag=on  DiscreDampingValue=DeviceDiscreDamping{25}  LinearizationTimes=1  DirectFeedthrough=off
      settings: SourceProductName=Simplex Power Systems
  VSI-PLL26 : SimplexPS/Grid-Following Voltage-Source Inverter (dq-Frame System Object)  Ts=Ts  Sbase=Sbase  Vbase=Vbase  Wbase=Wbase  DeviceType=DeviceType{26}  DevicePara=DevicePara{26}  PowerFlow=DevicePowerFlow{26}  x0=x_e{26}  OtherInputs=OtherInputs{26}  DiscreMethod=Hybrid Trapezoidal  EnableInsideModification=off  DiscreDampingFlag=on  DiscreDampingValue=DeviceDiscreDamping{26}  LinearizationTimes=1  DirectFeedthrough=off
      settings: SourceProductName=Simplex Power Systems
  VSI-PLL27 : SimplexPS/Grid-Following Voltage-Source Inverter (dq-Frame System Object)  Ts=Ts  Sbase=Sbase  Vbase=Vbase  Wbase=Wbase  DeviceType=DeviceType{27}  DevicePara=DevicePara{27}  PowerFlow=DevicePowerFlow{27}  x0=x_e{27}  OtherInputs=OtherInputs{27}  DiscreMethod=Hybrid Trapezoidal  EnableInsideModification=off  DiscreDampingFlag=on  DiscreDampingValue=DeviceDiscreDamping{27}  LinearizationTimes=1  DirectFeedthrough=off
      settings: SourceProductName=Simplex Power Systems
  VSI-PLL28 : SimplexPS/Grid-Following Voltage-Source Inverter (dq-Frame System Object)  Ts=Ts  Sbase=Sbase  Vbase=Vbase  Wbase=Wbase  DeviceType=DeviceType{28}  DevicePara=DevicePara{28}  PowerFlow=DevicePowerFlow{28}  x0=x_e{28}  OtherInputs=OtherInputs{28}  DiscreMethod=Hybrid Trapezoidal  EnableInsideModification=off  DiscreDampingFlag=on  DiscreDampingValue=DeviceDiscreDamping{28}  LinearizationTimes=1  DirectFeedthrough=off
      settings: SourceProductName=Simplex Power Systems
  VSI-PLL29 : SimplexPS/Grid-Following Voltage-Source Inverter (dq-Frame System Object)  Ts=Ts  Sbase=Sbase  Vbase=Vbase  Wbase=Wbase  DeviceType=DeviceType{29}  DevicePara=DevicePara{29}  PowerFlow=DevicePowerFlow{29}  x0=x_e{29}  OtherInputs=OtherInputs{29}  DiscreMethod=Hybrid Trapezoidal  EnableInsideModification=off  DiscreDampingFlag=on  DiscreDampingValue=DeviceDiscreDamping{29}  LinearizationTimes=1  DirectFeedthrough=off
      settings: SourceProductName=Simplex Power Systems
  VSI-PLL3 : SimplexPS/Grid-Following Voltage-Source Inverter (dq-Frame System Object)  Ts=Ts  Sbase=Sbase  Vbase=Vbase  Wbase=Wbase  DeviceType=DeviceType{3}  DevicePara=DevicePara{3}  PowerFlow=DevicePowerFlow{3}  x0=x_e{3}  OtherInputs=OtherInputs{3}  DiscreMethod=Hybrid Trapezoidal  EnableInsideModification=off  DiscreDampingFlag=on  DiscreDampingValue=DeviceDiscreDamping{3}  LinearizationTimes=1  DirectFeedthrough=off
      settings: SourceProductName=Simplex Power Systems
  VSI-PLL33 : SimplexPS/Grid-Following Voltage-Source Inverter (dq-Frame System Object)  Ts=Ts  Sbase=Sbase  Vbase=Vbase  Wbase=Wbase  DeviceType=DeviceType{33}  DevicePara=DevicePara{33}  PowerFlow=DevicePowerFlow{33}  x0=x_e{33}  OtherInputs=OtherInputs{33}  DiscreMethod=Hybrid Trapezoidal  EnableInsideModification=off  DiscreDampingFlag=on  DiscreDampingValue=DeviceDiscreDamping{33}  LinearizationTimes=1  DirectFeedthrough=off
      settings: SourceProductName=Simplex Power Systems
  VSI-PLL36 : SimplexPS/Grid-Following Voltage-Source Inverter (dq-Frame System Object)  Ts=Ts  Sbase=Sbase  Vbase=Vbase  Wbase=Wbase  DeviceType=DeviceType{36}  DevicePara=DevicePara{36}  PowerFlow=DevicePowerFlow{36}  x0=x_e{36}  OtherInputs=OtherInputs{36}  DiscreMethod=Hybrid Trapezoidal  EnableInsideModification=off  DiscreDampingFlag=on  DiscreDampingValue=DeviceDiscreDamping{36}  LinearizationTimes=1  DirectFeedthrough=off
      settings: SourceProductName=Simplex Power Systems
  VSI-PLL39 : SimplexPS/Grid-Following Voltage-Source Inverter (dq-Frame System Object)  Ts=Ts  Sbase=Sbase  Vbase=Vbase  Wbase=Wbase  DeviceType=DeviceType{39}  DevicePara=DevicePara{39}  PowerFlow=DevicePowerFlow{39}  x0=x_e{39}  OtherInputs=OtherInputs{39}  DiscreMethod=Hybrid Trapezoidal  EnableInsideModification=off  DiscreDampingFlag=on  DiscreDampingValue=DeviceDiscreDamping{39}  LinearizationTimes=1  DirectFeedthrough=off
      settings: SourceProductName=Simplex Power Systems
  VSI-PLL4 : SimplexPS/Grid-Following Voltage-Source Inverter (dq-Frame System Object)  Ts=Ts  Sbase=Sbase  Vbase=Vbase  Wbase=Wbase  DeviceType=DeviceType{4}  DevicePara=DevicePara{4}  PowerFlow=DevicePowerFlow{4}  x0=x_e{4}  OtherInputs=OtherInputs{4}  DiscreMethod=Hybrid Trapezoidal  EnableInsideModification=off  DiscreDampingFlag=on  DiscreDampingValue=DeviceDiscreDamping{4}  LinearizationTimes=1  DirectFeedthrough=off
      settings: SourceProductName=Simplex Power Systems
  VSI-PLL40 : SimplexPS/Grid-Following Voltage-Source Inverter (dq-Frame System Object)  Ts=Ts  Sbase=Sbase  Vbase=Vbase  Wbase=Wbase  DeviceType=DeviceType{40}  DevicePara=DevicePara{40}  PowerFlow=DevicePowerFlow{40}  x0=x_e{40}  OtherInputs=OtherInputs{40}  DiscreMethod=Hybrid Trapezoidal  EnableInsideModification=off  DiscreDampingFlag=on  DiscreDampingValue=DeviceDiscreDamping{40}  LinearizationTimes=1  DirectFeedthrough=off
      settings: SourceProductName=Simplex Power Systems
  VSI-PLL41 : SimplexPS/Grid-Following Voltage-Source Inverter (dq-Frame System Object)  Ts=Ts  Sbase=Sbase  Vbase=Vbase  Wbase=Wbase  DeviceType=DeviceType{41}  DevicePara=DevicePara{41}  PowerFlow=DevicePowerFlow{41}  x0=x_e{41}  OtherInputs=OtherInputs{41}  DiscreMethod=Hybrid Trapezoidal  EnableInsideModification=off  DiscreDampingFlag=on  DiscreDampingValue=DeviceDiscreDamping{41}  LinearizationTimes=1  DirectFeedthrough=off
      settings: SourceProductName=Simplex Power Systems
  VSI-PLL42 : SimplexPS/Grid-Following Voltage-Source Inverter (dq-Frame System Object)  Ts=Ts  Sbase=Sbase  Vbase=Vbase  Wbase=Wbase  DeviceType=DeviceType{42}  DevicePara=DevicePara{42}  PowerFlow=DevicePowerFlow{42}  x0=x_e{42}  OtherInputs=OtherInputs{42}  DiscreMethod=Hybrid Trapezoidal  EnableInsideModification=off  DiscreDampingFlag=on  DiscreDampingValue=DeviceDiscreDamping{42}  LinearizationTimes=1  DirectFeedthrough=off
      settings: SourceProductName=Simplex Power Systems
  VSI-PLL44 : SimplexPS/Grid-Following Voltage-Source Inverter (dq-Frame System Object)  Ts=Ts  Sbase=Sbase  Vbase=Vbase  Wbase=Wbase  DeviceType=DeviceType{44}  DevicePara=DevicePara{44}  PowerFlow=DevicePowerFlow{44}  x0=x_e{44}  OtherInputs=OtherInputs{44}  DiscreMethod=Hybrid Trapezoidal  EnableInsideModification=off  DiscreDampingFlag=on  DiscreDampingValue=DeviceDiscreDamping{44}  LinearizationTimes=1  DirectFeedthrough=off
      settings: SourceProductName=Simplex Power Systems
  VSI-PLL45 : SimplexPS/Grid-Following Voltage-Source Inverter (dq-Frame System Object)  Ts=Ts  Sbase=Sbase  Vbase=Vbase  Wbase=Wbase  DeviceType=DeviceType{45}  DevicePara=DevicePara{45}  PowerFlow=DevicePowerFlow{45}  x0=x_e{45}  OtherInputs=OtherInputs{45}  DiscreMethod=Hybrid Trapezoidal  EnableInsideModification=off  DiscreDampingFlag=on  DiscreDampingValue=DeviceDiscreDamping{45}  LinearizationTimes=1  DirectFeedthrough=off
      settings: SourceProductName=Simplex Power Systems
  VSI-PLL46 : SimplexPS/Grid-Following Voltage-Source Inverter (dq-Frame System Object)  Ts=Ts  Sbase=Sbase  Vbase=Vbase  Wbase=Wbase  DeviceType=DeviceType{46}  DevicePara=DevicePara{46}  PowerFlow=DevicePowerFlow{46}  x0=x_e{46}  OtherInputs=OtherInputs{46}  DiscreMethod=Hybrid Trapezoidal  EnableInsideModification=off  DiscreDampingFlag=on  DiscreDampingValue=DeviceDiscreDamping{46}  LinearizationTimes=1  DirectFeedthrough=off
      settings: SourceProductName=Simplex Power Systems
  VSI-PLL47 : SimplexPS/Grid-Following Voltage-Source Inverter (dq-Frame System Object)  Ts=Ts  Sbase=Sbase  Vbase=Vbase  Wbase=Wbase  DeviceType=DeviceType{47}  DevicePara=DevicePara{47}  PowerFlow=DevicePowerFlow{47}  x0=x_e{47}  OtherInputs=OtherInputs{47}  DiscreMethod=Hybrid Trapezoidal  EnableInsideModification=off  DiscreDampingFlag=on  DiscreDampingValue=DeviceDiscreDamping{47}  LinearizationTimes=1  DirectFeedthrough=off
      settings: SourceProductName=Simplex Power Systems
  VSI-PLL48 : SimplexPS/Grid-Following Voltage-Source Inverter (dq-Frame System Object)  Ts=Ts  Sbase=Sbase  Vbase=Vbase  Wbase=Wbase  DeviceType=DeviceType{48}  DevicePara=DevicePara{48}  PowerFlow=DevicePowerFlow{48}  x0=x_e{48}  OtherInputs=OtherInputs{48}  DiscreMethod=Hybrid Trapezoidal  EnableInsideModification=off  DiscreDampingFlag=on  DiscreDampingValue=DeviceDiscreDamping{48}  LinearizationTimes=1  DirectFeedthrough=off
      settings: SourceProductName=Simplex Power Systems
  VSI-PLL49 : SimplexPS/Grid-Following Voltage-Source Inverter (dq-Frame System Object)  Ts=Ts  Sbase=Sbase  Vbase=Vbase  Wbase=Wbase  DeviceType=DeviceType{49}  DevicePara=DevicePara{49}  PowerFlow=DevicePowerFlow{49}  x0=x_e{49}  OtherInputs=OtherInputs{49}  DiscreMethod=Hybrid Trapezoidal  EnableInsideModification=off  DiscreDampingFlag=on  DiscreDampingValue=DeviceDiscreDamping{49}  LinearizationTimes=1  DirectFeedthrough=off
      settings: SourceProductName=Simplex Power Systems
  VSI-PLL5 : SimplexPS/Grid-Following Voltage-Source Inverter (dq-Frame System Object)  Ts=Ts  Sbase=Sbase  Vbase=Vbase  Wbase=Wbase  DeviceType=DeviceType{5}  DevicePara=DevicePara{5}  PowerFlow=DevicePowerFlow{5}  x0=x_e{5}  OtherInputs=OtherInputs{5}  DiscreMethod=Hybrid Trapezoidal  EnableInsideModification=off  DiscreDampingFlag=on  DiscreDampingValue=DeviceDiscreDamping{5}  LinearizationTimes=1  DirectFeedthrough=off
      settings: SourceProductName=Simplex Power Systems
  VSI-PLL50 : SimplexPS/Grid-Following Voltage-Source Inverter (dq-Frame System Object)  Ts=Ts  Sbase=Sbase  Vbase=Vbase  Wbase=Wbase  DeviceType=DeviceType{50}  DevicePara=DevicePara{50}  PowerFlow=DevicePowerFlow{50}  x0=x_e{50}  OtherInputs=OtherInputs{50}  DiscreMethod=Hybrid Trapezoidal  EnableInsideModification=off  DiscreDampingFlag=on  DiscreDampingValue=DeviceDiscreDamping{50}  LinearizationTimes=1  DirectFeedthrough=off
      settings: SourceProductName=Simplex Power Systems
  VSI-PLL51 : SimplexPS/Grid-Following Voltage-Source Inverter (dq-Frame System Object)  Ts=Ts  Sbase=Sbase  Vbase=Vbase  Wbase=Wbase  DeviceType=DeviceType{51}  DevicePara=DevicePara{51}  PowerFlow=DevicePowerFlow{51}  x0=x_e{51}  OtherInputs=OtherInputs{51}  DiscreMethod=Hybrid Trapezoidal  EnableInsideModification=off  DiscreDampingFlag=on  DiscreDampingValue=DeviceDiscreDamping{51}  LinearizationTimes=1  DirectFeedthrough=off
      settings: SourceProductName=Simplex Power Systems
  VSI-PLL52 : SimplexPS/Grid-Following Voltage-Source Inverter (dq-Frame System Object)  Ts=Ts  Sbase=Sbase  Vbase=Vbase  Wbase=Wbase  DeviceType=DeviceType{52}  DevicePara=DevicePara{52}  PowerFlow=DevicePowerFlow{52}  x0=x_e{52}  OtherInputs=OtherInputs{52}  DiscreMethod=Hybrid Trapezoidal  EnableInsideModification=off  DiscreDampingFlag=on  DiscreDampingValue=DeviceDiscreDamping{52}  LinearizationTimes=1  DirectFeedthrough=off
      settings: SourceProductName=Simplex Power Systems
  VSI-PLL53 : SimplexPS/Grid-Following Voltage-Source Inverter (dq-Frame System Object)  Ts=Ts  Sbase=Sbase  Vbase=Vbase  Wbase=Wbase  DeviceType=DeviceType{53}  DevicePara=DevicePara{53}  PowerFlow=DevicePowerFlow{53}  x0=x_e{53}  OtherInputs=OtherInputs{53}  DiscreMethod=Hybrid Trapezoidal  EnableInsideModification=off  DiscreDampingFlag=on  DiscreDampingValue=DeviceDiscreDamping{53}  LinearizationTimes=1  DirectFeedthrough=off
      settings: SourceProductName=Simplex Power Systems
  VSI-PLL55 : SimplexPS/Grid-Following Voltage-Source Inverter (dq-Frame System Object)  Ts=Ts  Sbase=Sbase  Vbase=Vbase  Wbase=Wbase  DeviceType=DeviceType{55}  DevicePara=DevicePara{55}  PowerFlow=DevicePowerFlow{55}  x0=x_e{55}  OtherInputs=OtherInputs{55}  DiscreMethod=Hybrid Trapezoidal  EnableInsideModification=off  DiscreDampingFlag=on  DiscreDampingValue=DeviceDiscreDamping{55}  LinearizationTimes=1  DirectFeedthrough=off
      settings: SourceProductName=Simplex Power Systems
  VSI-PLL56 : SimplexPS/Grid-Following Voltage-Source Inverter (dq-Frame System Object)  Ts=Ts  Sbase=Sbase  Vbase=Vbase  Wbase=Wbase  DeviceType=DeviceType{56}  DevicePara=DevicePara{56}  PowerFlow=DevicePowerFlow{56}  x0=x_e{56}  OtherInputs=OtherInputs{56}  DiscreMethod=Hybrid Trapezoidal  EnableInsideModification=off  DiscreDampingFlag=on  DiscreDampingValue=DeviceDiscreDamping{56}  LinearizationTimes=1  DirectFeedthrough=off
      settings: SourceProductName=Simplex Power Systems
  VSI-PLL59 : SimplexPS/Grid-Following Voltage-Source Inverter (dq-Frame System Object)  Ts=Ts  Sbase=Sbase  Vbase=Vbase  Wbase=Wbase  DeviceType=DeviceType{59}  DevicePara=DevicePara{59}  PowerFlow=DevicePowerFlow{59}  x0=x_e{59}  OtherInputs=OtherInputs{59}  DiscreMethod=Hybrid Trapezoidal  EnableInsideModification=off  DiscreDampingFlag=on  DiscreDampingValue=DeviceDiscreDamping{59}  LinearizationTimes=1  DirectFeedthrough=off
      settings: SourceProductName=Simplex Power Systems
  VSI-PLL6 : SimplexPS/Grid-Following Voltage-Source Inverter (dq-Frame System Object)  Ts=Ts  Sbase=Sbase  Vbase=Vbase  Wbase=Wbase  DeviceType=DeviceType{6}  DevicePara=DevicePara{6}  PowerFlow=DevicePowerFlow{6}  x0=x_e{6}  OtherInputs=OtherInputs{6}  DiscreMethod=Hybrid Trapezoidal  EnableInsideModification=off  DiscreDampingFlag=on  DiscreDampingValue=DeviceDiscreDamping{6}  LinearizationTimes=1  DirectFeedthrough=off
      settings: SourceProductName=Simplex Power Systems
  VSI-PLL60 : SimplexPS/Grid-Following Voltage-Source Inverter (dq-Frame System Object)  Ts=Ts  Sbase=Sbase  Vbase=Vbase  Wbase=Wbase  DeviceType=DeviceType{60}  DevicePara=DevicePara{60}  PowerFlow=DevicePowerFlow{60}  x0=x_e{60}  OtherInputs=OtherInputs{60}  DiscreMethod=Hybrid Trapezoidal  EnableInsideModification=off  DiscreDampingFlag=on  DiscreDampingValue=DeviceDiscreDamping{60}  LinearizationTimes=1  DirectFeedthrough=off
      settings: SourceProductName=Simplex Power Systems
  VSI-PLL61 : SimplexPS/Grid-Following Voltage-Source Inverter (dq-Frame System Object)  Ts=Ts  Sbase=Sbase  Vbase=Vbase  Wbase=Wbase  DeviceType=DeviceType{61}  DevicePara=DevicePara{61}  PowerFlow=DevicePowerFlow{61}  x0=x_e{61}  OtherInputs=OtherInputs{61}  DiscreMethod=Hybrid Trapezoidal  EnableInsideModification=off  DiscreDampingFlag=on  DiscreDampingValue=DeviceDiscreDamping{61}  LinearizationTimes=1  DirectFeedthrough=off
      settings: SourceProductName=Simplex Power Systems
  VSI-PLL64 : SimplexPS/Grid-Following Voltage-Source Inverter (dq-Frame System Object)  Ts=Ts  Sbase=Sbase  Vbase=Vbase  Wbase=Wbase  DeviceType=DeviceType{64}  DevicePara=DevicePara{64}  PowerFlow=DevicePowerFlow{64}  x0=x_e{64}  OtherInputs=OtherInputs{64}  DiscreMethod=Hybrid Trapezoidal  EnableInsideModification=off  DiscreDampingFlag=on  DiscreDampingValue=DeviceDiscreDamping{64}  LinearizationTimes=1  DirectFeedthrough=off
      settings: SourceProductName=Simplex Power Systems
  VSI-PLL67 : SimplexPS/Grid-Following Voltage-Source Inverter (dq-Frame System Object)  Ts=Ts  Sbase=Sbase  Vbase=Vbase  Wbase=Wbase  DeviceType=DeviceType{67}  DevicePara=DevicePara{67}  PowerFlow=DevicePowerFlow{67}  x0=x_e{67}  OtherInputs=OtherInputs{67}  DiscreMethod=Hybrid Trapezoidal  EnableInsideModification=off  DiscreDampingFlag=on  DiscreDampingValue=DeviceDiscreDamping{67}  LinearizationTimes=1  DirectFeedthrough=off
      settings: SourceProductName=Simplex Power Systems
  VSI-PLL68 : SimplexPS/Grid-Following Voltage-Source Inverter (dq-Frame System Object)  Ts=Ts  Sbase=Sbase  Vbase=Vbase  Wbase=Wbase  DeviceType=DeviceType{68}  DevicePara=DevicePara{68}  PowerFlow=DevicePowerFlow{68}  x0=x_e{68}  OtherInputs=OtherInputs{68}  DiscreMethod=Hybrid Trapezoidal  EnableInsideModification=off  DiscreDampingFlag=on  DiscreDampingValue=DeviceDiscreDamping{68}  LinearizationTimes=1  DirectFeedthrough=off
      settings: SourceProductName=Simplex Power Systems
  VSI-PLL7 : SimplexPS/Grid-Following Voltage-Source Inverter (dq-Frame System Object)  Ts=Ts  Sbase=Sbase  Vbase=Vbase  Wbase=Wbase  DeviceType=DeviceType{7}  DevicePara=DevicePara{7}  PowerFlow=DevicePowerFlow{7}  x0=x_e{7}  OtherInputs=OtherInputs{7}  DiscreMethod=Hybrid Trapezoidal  EnableInsideModification=off  DiscreDampingFlag=on  DiscreDampingValue=DeviceDiscreDamping{7}  LinearizationTimes=1  DirectFeedthrough=off
      settings: SourceProductName=Simplex Power Systems
  VSI-PLL8 : SimplexPS/Grid-Following Voltage-Source Inverter (dq-Frame System Object)  Ts=Ts  Sbase=Sbase  Vbase=Vbase  Wbase=Wbase  DeviceType=DeviceType{8}  DevicePara=DevicePara{8}  PowerFlow=DevicePowerFlow{8}  x0=x_e{8}  OtherInputs=OtherInputs{8}  DiscreMethod=Hybrid Trapezoidal  EnableInsideModification=off  DiscreDampingFlag=on  DiscreDampingValue=DeviceDiscreDamping{8}  LinearizationTimes=1  DirectFeedthrough=off
      settings: SourceProductName=Simplex Power Systems
  VSI-PLL9 : SimplexPS/Grid-Following Voltage-Source Inverter (dq-Frame System Object)  Ts=Ts  Sbase=Sbase  Vbase=Vbase  Wbase=Wbase  DeviceType=DeviceType{9}  DevicePara=DevicePara{9}  PowerFlow=DevicePowerFlow{9}  x0=x_e{9}  OtherInputs=OtherInputs{9}  DiscreMethod=Hybrid Trapezoidal  EnableInsideModification=off  DiscreDampingFlag=on  DiscreDampingValue=DeviceDiscreDamping{9}  LinearizationTimes=1  DirectFeedthrough=off
      settings: SourceProductName=Simplex Power Systems
  powergui : powerlib/powergui  Priority=1  SimulationMode=Discrete  SampleTime=Ts  frequency=60  Iterations=50  frequencyindice=0  Pbase=100e6  ErrMax=1e-4  UnitsV=kV  UnitsW=MW  buscounter=0  FunctionMessages=off  echomessages=off  EnableUseOfTLC=off  CurrentSourceSwitches=off  DisableSnubberDevices=off  DisableRonSwitches=off  DisableVfSwitches=off  DisplayEquations=off  AutomaticDiscreteSolvers=off  SolverType=Tustin/Backward Euler (TBE)  Interpol=off  ExternalGateDelay=off  methode=off  Ts=100  x0status=blocks  SPID=on  SwTol=0  HookPort=off  NonlinearTolerance=1e-4  nMaxIteration=100  ContinueOnMaxIteration=off  RestoreLinks=warning  ResistiveCurrentMeasurement=off  Frange=[0:2:500]  Ylog=off  Xlog=on  ShowGrid=off  save=off  variable=ZData  structure=0  ZoomFFT=off  StartTime=0.0  cycles=1  DisplayStyle=1  fundamental=60  FreqAxis=off  MaxFrequency=1000  frequencyindicesteady=1  RmsSteady=1  display=off
  wires:
  VSI-PLL1/1 -> DS-Bus1/1
  DS-Bus1/1 -> D-Scope1/1  "<v_dq>"
  DS-Bus1/2 -> D-Scope1/2  "<i_dq>"
  DS-Bus1/3 -> D-Scope1/3  "<v_abc>"
  DS-Bus1/4 -> D-Scope1/4  "<i_abc>"
  DS-Bus1/5 -> D-Scope1/5  "<w>"
  DS-Bus1/6 -> D-Scope1/6  "<theta>"
  DS-Bus1/7 -> D-Scope1/7  "<pq>"
  VSI-PLL2/1 -> DS-Bus2/1
  DS-Bus2/1 -> D-Scope2/1  "<v_dq>"
  DS-Bus2/2 -> D-Scope2/2  "<i_dq>"
  DS-Bus2/3 -> D-Scope2/3  "<v_abc>"
  DS-Bus2/4 -> D-Scope2/4  "<i_abc>"
  DS-Bus2/5 -> D-Scope2/5  "<w>"
  DS-Bus2/6 -> D-Scope2/6  "<theta>"
  DS-Bus2/7 -> D-Scope2/7  "<pq>"
  VSI-PLL3/1 -> DS-Bus3/1
  DS-Bus3/1 -> D-Scope3/1  "<v_dq>"
  DS-Bus3/2 -> D-Scope3/2  "<i_dq>"
  DS-Bus3/3 -> D-Scope3/3  "<v_abc>"
  DS-Bus3/4 -> D-Scope3/4  "<i_abc>"
  DS-Bus3/5 -> D-Scope3/5  "<w>"
  DS-Bus3/6 -> D-Scope3/6  "<theta>"
  DS-Bus3/7 -> D-Scope3/7  "<pq>"
  VSI-PLL4/1 -> DS-Bus4/1
  DS-Bus4/1 -> D-Scope4/1  "<v_dq>"
  DS-Bus4/2 -> D-Scope4/2  "<i_dq>"
  DS-Bus4/3 -> D-Scope4/3  "<v_abc>"
  DS-Bus4/4 -> D-Scope4/4  "<i_abc>"
  DS-Bus4/5 -> D-Scope4/5  "<w>"
  DS-Bus4/6 -> D-Scope4/6  "<theta>"
  DS-Bus4/7 -> D-Scope4/7  "<pq>"
  VSI-PLL5/1 -> DS-Bus5/1
  DS-Bus5/1 -> D-Scope5/1  "<v_dq>"
  DS-Bus5/2 -> D-Scope5/2  "<i_dq>"
  DS-Bus5/3 -> D-Scope5/3  "<v_abc>"
  DS-Bus5/4 -> D-Scope5/4  "<i_abc>"
  DS-Bus5/5 -> D-Scope5/5  "<w>"
  DS-Bus5/6 -> D-Scope5/6  "<theta>"
  DS-Bus5/7 -> D-Scope5/7  "<pq>"
  VSI-PLL6/1 -> DS-Bus6/1
  DS-Bus6/1 -> D-Scope6/1  "<v_dq>"
  DS-Bus6/2 -> D-Scope6/2  "<i_dq>"
  DS-Bus6/3 -> D-Scope6/3  "<v_abc>"
  DS-Bus6/4 -> D-Scope6/4  "<i_abc>"
  DS-Bus6/5 -> D-Scope6/5  "<w>"
  DS-Bus6/6 -> D-Scope6/6  "<theta>"
  DS-Bus6/7 -> D-Scope6/7  "<pq>"
  VSI-PLL7/1 -> DS-Bus7/1
  DS-Bus7/1 -> D-Scope7/1  "<v_dq>"
  DS-Bus7/2 -> D-Scope7/2  "<i_dq>"
  DS-Bus7/3 -> D-Scope7/3  "<v_abc>"
  DS-Bus7/4 -> D-Scope7/4  "<i_abc>"
  DS-Bus7/5 -> D-Scope7/5  "<w>"
  DS-Bus7/6 -> D-Scope7/6  "<theta>"
  DS-Bus7/7 -> D-Scope7/7  "<pq>"
  VSI-PLL8/1 -> DS-Bus8/1
  DS-Bus8/1 -> D-Scope8/1  "<v_dq>"
  DS-Bus8/2 -> D-Scope8/2  "<i_dq>"
  DS-Bus8/3 -> D-Scope8/3  "<v_abc>"
  DS-Bus8/4 -> D-Scope8/4  "<i_abc>"
  DS-Bus8/5 -> D-Scope8/5  "<w>"
  DS-Bus8/6 -> D-Scope8/6  "<theta>"
  DS-Bus8/7 -> D-Scope8/7  "<pq>"
  VSI-PLL9/1 -> DS-Bus9/1
  DS-Bus9/1 -> D-Scope9/1  "<v_dq>"
  DS-Bus9/2 -> D-Scope9/2  "<i_dq>"
  DS-Bus9/3 -> D-Scope9/3  "<v_abc>"
  DS-Bus9/4 -> D-Scope9/4  "<i_abc>"
  DS-Bus9/5 -> D-Scope9/5  "<w>"
  DS-Bus9/6 -> D-Scope9/6  "<theta>"
  DS-Bus9/7 -> D-Scope9/7  "<pq>"
  VSI-PLL10/1 -> DS-Bus10/1
  DS-Bus10/1 -> D-Scope10/1  "<v_dq>"
  DS-Bus10/2 -> D-Scope10/2  "<i_dq>"
  DS-Bus10/3 -> D-Scope10/3  "<v_abc>"
  DS-Bus10/4 -> D-Scope10/4  "<i_abc>"
  DS-Bus10/5 -> D-Scope10/5  "<w>"
  DS-Bus10/6 -> D-Scope10/6  "<theta>"
  DS-Bus10/7 -> D-Scope10/7  "<pq>"
  VSI-PLL11/1 -> DS-Bus11/1
  DS-Bus11/1 -> D-Scope11/1  "<v_dq>"
  DS-Bus11/2 -> D-Scope11/2  "<i_dq>"
  DS-Bus11/3 -> D-Scope11/3  "<v_abc>"
  DS-Bus11/4 -> D-Scope11/4  "<i_abc>"
  DS-Bus11/5 -> D-Scope11/5  "<w>"
  DS-Bus11/6 -> D-Scope11/6  "<theta>"
  DS-Bus11/7 -> D-Scope11/7  "<pq>"
  VSI-PLL12/1 -> DS-Bus12/1
  DS-Bus12/1 -> D-Scope12/1  "<v_dq>"
  DS-Bus12/2 -> D-Scope12/2  "<i_dq>"
  DS-Bus12/3 -> D-Scope12/3  "<v_abc>"
  DS-Bus12/4 -> D-Scope12/4  "<i_abc>"
  DS-Bus12/5 -> D-Scope12/5  "<w>"
  DS-Bus12/6 -> D-Scope12/6  "<theta>"
  DS-Bus12/7 -> D-Scope12/7  "<pq>"
  VSI-PLL13/1 -> DS-Bus13/1
  DS-Bus13/1 -> D-Scope13/1  "<v_dq>"
  DS-Bus13/2 -> D-Scope13/2  "<i_dq>"
  DS-Bus13/3 -> D-Scope13/3  "<v_abc>"
  DS-Bus13/4 -> D-Scope13/4  "<i_abc>"
  DS-Bus13/5 -> D-Scope13/5  "<w>"
  DS-Bus13/6 -> D-Scope13/6  "<theta>"
  DS-Bus13/7 -> D-Scope13/7  "<pq>"
  VSI-PLL14/1 -> DS-Bus14/1
  DS-Bus14/1 -> D-Scope14/1  "<v_dq>"
  DS-Bus14/2 -> D-Scope14/2  "<i_dq>"
  DS-Bus14/3 -> D-Scope14/3  "<v_abc>"
  DS-Bus14/4 -> D-Scope14/4  "<i_abc>"
  DS-Bus14/5 -> D-Scope14/5  "<w>"
  DS-Bus14/6 -> D-Scope14/6  "<theta>"
  DS-Bus14/7 -> D-Scope14/7  "<pq>"
  VSI-PLL15/1 -> DS-Bus15/1
  DS-Bus15/1 -> D-Scope15/1  "<v_dq>"
  DS-Bus15/2 -> D-Scope15/2  "<i_dq>"
  DS-Bus15/3 -> D-Scope15/3  "<v_abc>"
  DS-Bus15/4 -> D-Scope15/4  "<i_abc>"
  DS-Bus15/5 -> D-Scope15/5  "<w>"
  DS-Bus15/6 -> D-Scope15/6  "<theta>"
  DS-Bus15/7 -> D-Scope15/7  "<pq>"
  VSI-PLL16/1 -> DS-Bus16/1
  DS-Bus16/1 -> D-Scope16/1  "<v_dq>"
  DS-Bus16/2 -> D-Scope16/2  "<i_dq>"
  DS-Bus16/3 -> D-Scope16/3  "<v_abc>"
  DS-Bus16/4 -> D-Scope16/4  "<i_abc>"
  DS-Bus16/5 -> D-Scope16/5  "<w>"
  DS-Bus16/6 -> D-Scope16/6  "<theta>"
  DS-Bus16/7 -> D-Scope16/7  "<pq>"
  VSI-PLL17/1 -> DS-Bus17/1
  DS-Bus17/1 -> D-Scope17/1  "<v_dq>"
  DS-Bus17/2 -> D-Scope17/2  "<i_dq>"
  DS-Bus17/3 -> D-Scope17/3  "<v_abc>"
  DS-Bus17/4 -> D-Scope17/4  "<i_abc>"
  DS-Bus17/5 -> D-Scope17/5  "<w>"
  DS-Bus17/6 -> D-Scope17/6  "<theta>"
  DS-Bus17/7 -> D-Scope17/7  "<pq>"
  VSI-PLL18/1 -> DS-Bus18/1
  DS-Bus18/1 -> D-Scope18/1  "<v_dq>"
  DS-Bus18/2 -> D-Scope18/2  "<i_dq>"
  DS-Bus18/3 -> D-Scope18/3  "<v_abc>"
  DS-Bus18/4 -> D-Scope18/4  "<i_abc>"
  DS-Bus18/5 -> D-Scope18/5  "<w>"
  DS-Bus18/6 -> D-Scope18/6  "<theta>"
  DS-Bus18/7 -> D-Scope18/7  "<pq>"
  VSI-PLL20/1 -> DS-Bus20/1
  DS-Bus20/1 -> D-Scope20/1  "<v_dq>"
  DS-Bus20/2 -> D-Scope20/2  "<i_dq>"
  DS-Bus20/3 -> D-Scope20/3  "<v_abc>"
  DS-Bus20/4 -> D-Scope20/4  "<i_abc>"
  DS-Bus20/5 -> D-Scope20/5  "<w>"
  DS-Bus20/6 -> D-Scope20/6  "<theta>"
  DS-Bus20/7 -> D-Scope20/7  "<pq>"
  VSI-PLL21/1 -> DS-Bus21/1
  DS-Bus21/1 -> D-Scope21/1  "<v_dq>"
  DS-Bus21/2 -> D-Scope21/2  "<i_dq>"
  DS-Bus21/3 -> D-Scope21/3  "<v_abc>"
  DS-Bus21/4 -> D-Scope21/4  "<i_abc>"
  DS-Bus21/5 -> D-Scope21/5  "<w>"
  DS-Bus21/6 -> D-Scope21/6  "<theta>"
  DS-Bus21/7 -> D-Scope21/7  "<pq>"
  VSI-PLL23/1 -> DS-Bus23/1
  DS-Bus23/1 -> D-Scope23/1  "<v_dq>"
  DS-Bus23/2 -> D-Scope23/2  "<i_dq>"
  DS-Bus23/3 -> D-Scope23/3  "<v_abc>"
  DS-Bus23/4 -> D-Scope23/4  "<i_abc>"
  DS-Bus23/5 -> D-Scope23/5  "<w>"
  DS-Bus23/6 -> D-Scope23/6  "<theta>"
  DS-Bus23/7 -> D-Scope23/7  "<pq>"
  VSI-PLL24/1 -> DS-Bus24/1
  DS-Bus24/1 -> D-Scope24/1  "<v_dq>"
  DS-Bus24/2 -> D-Scope24/2  "<i_dq>"
  DS-Bus24/3 -> D-Scope24/3  "<v_abc>"
  DS-Bus24/4 -> D-Scope24/4  "<i_abc>"
  DS-Bus24/5 -> D-Scope24/5  "<w>"
  DS-Bus24/6 -> D-Scope24/6  "<theta>"
  DS-Bus24/7 -> D-Scope24/7  "<pq>"
  VSI-PLL25/1 -> DS-Bus25/1
  DS-Bus25/1 -> D-Scope25/1  "<v_dq>"
  DS-Bus25/2 -> D-Scope25/2  "<i_dq>"
  DS-Bus25/3 -> D-Scope25/3  "<v_abc>"
  DS-Bus25/4 -> D-Scope25/4  "<i_abc>"
  DS-Bus25/5 -> D-Scope25/5  "<w>"
  DS-Bus25/6 -> D-Scope25/6  "<theta>"
  DS-Bus25/7 -> D-Scope25/7  "<pq>"
  VSI-PLL26/1 -> DS-Bus26/1
  DS-Bus26/1 -> D-Scope26/1  "<v_dq>"
  DS-Bus26/2 -> D-Scope26/2  "<i_dq>"
  DS-Bus26/3 -> D-Scope26/3  "<v_abc>"
  DS-Bus26/4 -> D-Scope26/4  "<i_abc>"
  DS-Bus26/5 -> D-Scope26/5  "<w>"
  DS-Bus26/6 -> D-Scope26/6  "<theta>"
  DS-Bus26/7 -> D-Scope26/7  "<pq>"
  VSI-PLL27/1 -> DS-Bus27/1
  DS-Bus27/1 -> D-Scope27/1  "<v_dq>"
  DS-Bus27/2 -> D-Scope27/2  "<i_dq>"
  DS-Bus27/3 -> D-Scope27/3  "<v_abc>"
  DS-Bus27/4 -> D-Scope27/4  "<i_abc>"
  DS-Bus27/5 -> D-Scope27/5  "<w>"
  DS-Bus27/6 -> D-Scope27/6  "<theta>"
  DS-Bus27/7 -> D-Scope27/7  "<pq>"
  VSI-PLL28/1 -> DS-Bus28/1
  DS-Bus28/1 -> D-Scope28/1  "<v_dq>"
  DS-Bus28/2 -> D-Scope28/2  "<i_dq>"
  DS-Bus28/3 -> D-Scope28/3  "<v_abc>"
  DS-Bus28/4 -> D-Scope28/4  "<i_abc>"
  DS-Bus28/5 -> D-Scope28/5  "<w>"
  DS-Bus28/6 -> D-Scope28/6  "<theta>"
  DS-Bus28/7 -> D-Scope28/7  "<pq>"
  VSI-PLL29/1 -> DS-Bus29/1
  DS-Bus29/1 -> D-Scope29/1  "<v_dq>"
  DS-Bus29/2 -> D-Scope29/2  "<i_dq>"
  DS-Bus29/3 -> D-Scope29/3  "<v_abc>"
  DS-Bus29/4 -> D-Scope29/4  "<i_abc>"
  DS-Bus29/5 -> D-Scope29/5  "<w>"
  DS-Bus29/6 -> D-Scope29/6  "<theta>"
  DS-Bus29/7 -> D-Scope29/7  "<pq>"
  VSI-PLL33/1 -> DS-Bus33/1
  DS-Bus33/1 -> D-Scope33/1  "<v_dq>"
  DS-Bus33/2 -> D-Scope33/2  "<i_dq>"
  DS-Bus33/3 -> D-Scope33/3  "<v_abc>"
  DS-Bus33/4 -> D-Scope33/4  "<i_abc>"
  DS-Bus33/5 -> D-Scope33/5  "<w>"
  DS-Bus33/6 -> D-Scope33/6  "<theta>"
  DS-Bus33/7 -> D-Scope33/7  "<pq>"
  VSI-PLL36/1 -> DS-Bus36/1
  DS-Bus36/1 -> D-Scope36/1  "<v_dq>"
  DS-Bus36/2 -> D-Scope36/2  "<i_dq>"
  DS-Bus36/3 -> D-Scope36/3  "<v_abc>"
  DS-Bus36/4 -> D-Scope36/4  "<i_abc>"
  DS-Bus36/5 -> D-Scope36/5  "<w>"
  DS-Bus36/6 -> D-Scope36/6  "<theta>"
  DS-Bus36/7 -> D-Scope36/7  "<pq>"
  VSI-PLL39/1 -> DS-Bus39/1
  DS-Bus39/1 -> D-Scope39/1  "<v_dq>"
  DS-Bus39/2 -> D-Scope39/2  "<i_dq>"
  DS-Bus39/3 -> D-Scope39/3  "<v_abc>"
  DS-Bus39/4 -> D-Scope39/4  "<i_abc>"
  DS-Bus39/5 -> D-Scope39/5  "<w>"
  DS-Bus39/6 -> D-Scope39/6  "<theta>"
  DS-Bus39/7 -> D-Scope39/7  "<pq>"
  VSI-PLL40/1 -> DS-Bus40/1
  DS-Bus40/1 -> D-Scope40/1  "<v_dq>"
  DS-Bus40/2 -> D-Scope40/2  "<i_dq>"
  DS-Bus40/3 -> D-Scope40/3  "<v_abc>"
  DS-Bus40/4 -> D-Scope40/4  "<i_abc>"
  DS-Bus40/5 -> D-Scope40/5  "<w>"
  DS-Bus40/6 -> D-Scope40/6  "<theta>"
  DS-Bus40/7 -> D-Scope40/7  "<pq>"
  VSI-PLL41/1 -> DS-Bus41/1
  DS-Bus41/1 -> D-Scope41/1  "<v_dq>"
  DS-Bus41/2 -> D-Scope41/2  "<i_dq>"
  DS-Bus41/3 -> D-Scope41/3  "<v_abc>"
  DS-Bus41/4 -> D-Scope41/4  "<i_abc>"
  DS-Bus41/5 -> D-Scope41/5  "<w>"
  DS-Bus41/6 -> D-Scope41/6  "<theta>"
  DS-Bus41/7 -> D-Scope41/7  "<pq>"
  VSI-PLL42/1 -> DS-Bus42/1
  DS-Bus42/1 -> D-Scope42/1  "<v_dq>"
  DS-Bus42/2 -> D-Scope42/2  "<i_dq>"
  DS-Bus42/3 -> D-Scope42/3  "<v_abc>"
  DS-Bus42/4 -> D-Scope42/4  "<i_abc>"
  DS-Bus42/5 -> D-Scope42/5  "<w>"
  DS-Bus42/6 -> D-Scope42/6  "<theta>"
  DS-Bus42/7 -> D-Scope42/7  "<pq>"
  VSI-PLL44/1 -> DS-Bus44/1
  DS-Bus44/1 -> D-Scope44/1  "<v_dq>"
  DS-Bus44/2 -> D-Scope44/2  "<i_dq>"
  DS-Bus44/3 -> D-Scope44/3  "<v_abc>"
  DS-Bus44/4 -> D-Scope44/4  "<i_abc>"
  DS-Bus44/5 -> D-Scope44/5  "<w>"
  DS-Bus44/6 -> D-Scope44/6  "<theta>"
  DS-Bus44/7 -> D-Scope44/7  "<pq>"
  VSI-PLL45/1 -> DS-Bus45/1
  DS-Bus45/1 -> D-Scope45/1  "<v_dq>"
  DS-Bus45/2 -> D-Scope45/2  "<i_dq>"
  DS-Bus45/3 -> D-Scope45/3  "<v_abc>"
  DS-Bus45/4 -> D-Scope45/4  "<i_abc>"
  DS-Bus45/5 -> D-Scope45/5  "<w>"
  DS-Bus45/6 -> D-Scope45/6  "<theta>"
  DS-Bus45/7 -> D-Scope45/7  "<pq>"
  VSI-PLL46/1 -> DS-Bus46/1
  DS-Bus46/1 -> D-Scope46/1  "<v_dq>"
  DS-Bus46/2 -> D-Scope46/2  "<i_dq>"
  DS-Bus46/3 -> D-Scope46/3  "<v_abc>"
  DS-Bus46/4 -> D-Scope46/4  "<i_abc>"
  DS-Bus46/5 -> D-Scope46/5  "<w>"
  DS-Bus46/6 -> D-Scope46/6  "<theta>"
  DS-Bus46/7 -> D-Scope46/7  "<pq>"
  VSI-PLL47/1 -> DS-Bus47/1
  DS-Bus47/1 -> D-Scope47/1  "<v_dq>"
  DS-Bus47/2 -> D-Scope47/2  "<i_dq>"
  DS-Bus47/3 -> D-Scope47/3  "<v_abc>"
  DS-Bus47/4 -> D-Scope47/4  "<i_abc>"
  DS-Bus47/5 -> D-Scope47/5  "<w>"
  DS-Bus47/6 -> D-Scope47/6  "<theta>"
  DS-Bus47/7 -> D-Scope47/7  "<pq>"
  VSI-PLL48/1 -> DS-Bus48/1
  DS-Bus48/1 -> D-Scope48/1  "<v_dq>"
  DS-Bus48/2 -> D-Scope48/2  "<i_dq>"
  DS-Bus48/3 -> D-Scope48/3  "<v_abc>"
  DS-Bus48/4 -> D-Scope48/4  "<i_abc>"
  DS-Bus48/5 -> D-Scope48/5  "<w>"
  DS-Bus48/6 -> D-Scope48/6  "<theta>"
  DS-Bus48/7 -> D-Scope48/7  "<pq>"
  VSI-PLL49/1 -> DS-Bus49/1
  DS-Bus49/1 -> D-Scope49/1  "<v_dq>"
  DS-Bus49/2 -> D-Scope49/2  "<i_dq>"
  DS-Bus49/3 -> D-Scope49/3  "<v_abc>"
  DS-Bus49/4 -> D-Scope49/4  "<i_abc>"
  DS-Bus49/5 -> D-Scope49/5  "<w>"
  DS-Bus49/6 -> D-Scope49/6  "<theta>"
  DS-Bus49/7 -> D-Scope49/7  "<pq>"
  VSI-PLL50/1 -> DS-Bus50/1
  DS-Bus50/1 -> D-Scope50/1  "<v_dq>"
  DS-Bus50/2 -> D-Scope50/2  "<i_dq>"
  DS-Bus50/3 -> D-Scope50/3  "<v_abc>"
  DS-Bus50/4 -> D-Scope50/4  "<i_abc>"
  DS-Bus50/5 -> D-Scope50/5  "<w>"
  DS-Bus50/6 -> D-Scope50/6  "<theta>"
  DS-Bus50/7 -> D-Scope50/7  "<pq>"
  VSI-PLL51/1 -> DS-Bus51/1
  DS-Bus51/1 -> D-Scope51/1  "<v_dq>"
  DS-Bus51/2 -> D-Scope51/2  "<i_dq>"
  DS-Bus51/3 -> D-Scope51/3  "<v_abc>"
  DS-Bus51/4 -> D-Scope51/4  "<i_abc>"
  DS-Bus51/5 -> D-Scope51/5  "<w>"
  DS-Bus51/6 -> D-Scope51/6  "<theta>"
  DS-Bus51/7 -> D-Scope51/7  "<pq>"
  VSI-PLL52/1 -> DS-Bus52/1
  DS-Bus52/1 -> D-Scope52/1  "<v_dq>"
  DS-Bus52/2 -> D-Scope52/2  "<i_dq>"
  DS-Bus52/3 -> D-Scope52/3  "<v_abc>"
  DS-Bus52/4 -> D-Scope52/4  "<i_abc>"
  DS-Bus52/5 -> D-Scope52/5  "<w>"
  DS-Bus52/6 -> D-Scope52/6  "<theta>"
  DS-Bus52/7 -> D-Scope52/7  "<pq>"
  VSI-PLL53/1 -> DS-Bus53/1
  DS-Bus53/1 -> D-Scope53/1  "<v_dq>"
  DS-Bus53/2 -> D-Scope53/2  "<i_dq>"
  DS-Bus53/3 -> D-Scope53/3  "<v_abc>"
  DS-Bus53/4 -> D-Scope53/4  "<i_abc>"
  DS-Bus53/5 -> D-Scope53/5  "<w>"
  DS-Bus53/6 -> D-Scope53/6  "<theta>"
  DS-Bus53/7 -> D-Scope53/7  "<pq>"
  VSI-PLL55/1 -> DS-Bus55/1
  DS-Bus55/1 -> D-Scope55/1  "<v_dq>"
  DS-Bus55/2 -> D-Scope55/2  "<i_dq>"
  DS-Bus55/3 -> D-Scope55/3  "<v_abc>"
  DS-Bus55/4 -> D-Scope55/4  "<i_abc>"
  DS-Bus55/5 -> D-Scope55/5  "<w>"
  DS-Bus55/6 -> D-Scope55/6  "<theta>"
  DS-Bus55/7 -> D-Scope55/7  "<pq>"
  VSI-PLL56/1 -> DS-Bus56/1
  DS-Bus56/1 -> D-Scope56/1  "<v_dq>"
  DS-Bus56/2 -> D-Scope56/2  "<i_dq>"
  DS-Bus56/3 -> D-Scope56/3  "<v_abc>"
  DS-Bus56/4 -> D-Scope56/4  "<i_abc>"
  DS-Bus56/5 -> D-Scope56/5  "<w>"
  DS-Bus56/6 -> D-Scope56/6  "<theta>"
  DS-Bus56/7 -> D-Scope56/7  "<pq>"
  VSI-PLL59/1 -> DS-Bus59/1
  DS-Bus59/1 -> D-Scope59/1  "<v_dq>"
  DS-Bus59/2 -> D-Scope59/2  "<i_dq>"
  DS-Bus59/3 -> D-Scope59/3  "<v_abc>"
  DS-Bus59/4 -> D-Scope59/4  "<i_abc>"
  DS-Bus59/5 -> D-Scope59/5  "<w>"
  DS-Bus59/6 -> D-Scope59/6  "<theta>"
  DS-Bus59/7 -> D-Scope59/7  "<pq>"
  VSI-PLL60/1 -> DS-Bus60/1
  DS-Bus60/1 -> D-Scope60/1  "<v_dq>"
  DS-Bus60/2 -> D-Scope60/2  "<i_dq>"
  DS-Bus60/3 -> D-Scope60/3  "<v_abc>"
  DS-Bus60/4 -> D-Scope60/4  "<i_abc>"
  DS-Bus60/5 -> D-Scope60/5  "<w>"
  DS-Bus60/6 -> D-Scope60/6  "<theta>"
  DS-Bus60/7 -> D-Scope60/7  "<pq>"
  VSI-PLL61/1 -> DS-Bus61/1
  DS-Bus61/1 -> D-Scope61/1  "<v_dq>"
  DS-Bus61/2 -> D-Scope61/2  "<i_dq>"
  DS-Bus61/3 -> D-Scope61/3  "<v_abc>"
  DS-Bus61/4 -> D-Scope61/4  "<i_abc>"
  DS-Bus61/5 -> D-Scope61/5  "<w>"
  DS-Bus61/6 -> D-Scope61/6  "<theta>"
  DS-Bus61/7 -> D-Scope61/7  "<pq>"
  VSI-PLL64/1 -> DS-Bus64/1
  DS-Bus64/1 -> D-Scope64/1  "<v_dq>"
  DS-Bus64/2 -> D-Scope64/2  "<i_dq>"
  DS-Bus64/3 -> D-Scope64/3  "<v_abc>"
  DS-Bus64/4 -> D-Scope64/4  "<i_abc>"
  DS-Bus64/5 -> D-Scope64/5  "<w>"
  DS-Bus64/6 -> D-Scope64/6  "<theta>"
  DS-Bus64/7 -> D-Scope64/7  "<pq>"
  VSI-PLL67/1 -> DS-Bus67/1
  DS-Bus67/1 -> D-Scope67/1  "<v_dq>"
  DS-Bus67/2 -> D-Scope67/2  "<i_dq>"
  DS-Bus67/3 -> D-Scope67/3  "<v_abc>"
  DS-Bus67/4 -> D-Scope67/4  "<i_abc>"
  DS-Bus67/5 -> D-Scope67/5  "<w>"
  DS-Bus67/6 -> D-Scope67/6  "<theta>"
  DS-Bus67/7 -> D-Scope67/7  "<pq>"
  VSI-PLL68/1 -> DS-Bus68/1
  DS-Bus68/1 -> D-Scope68/1  "<v_dq>"
  DS-Bus68/2 -> D-Scope68/2  "<i_dq>"
  DS-Bus68/3 -> D-Scope68/3  "<v_abc>"
  DS-Bus68/4 -> D-Scope68/4  "<i_abc>"
  DS-Bus68/5 -> D-Scope68/5  "<w>"
  DS-Bus68/6 -> D-Scope68/6  "<theta>"
  DS-Bus68/7 -> D-Scope68/7  "<pq>"
  Current Measurement1/1 -> Scope1/1
  connections:
  VSI-PLL1/LConn4 -- D-GND1/LConn1
  VSI-PLL2/LConn4 -- D-GND2/LConn1
  VSI-PLL3/LConn4 -- D-GND3/LConn1
  VSI-PLL4/LConn4 -- D-GND4/LConn1
  VSI-PLL5/LConn4 -- D-GND5/LConn1
  VSI-PLL6/LConn4 -- D-GND6/LConn1
  VSI-PLL7/LConn4 -- D-GND7/LConn1
  VSI-PLL8/LConn4 -- D-GND8/LConn1
  VSI-PLL9/LConn4 -- D-GND9/LConn1
  VSI-PLL10/LConn4 -- D-GND10/LConn1
  VSI-PLL11/LConn4 -- D-GND11/LConn1
  VSI-PLL12/LConn4 -- D-GND12/LConn1
  VSI-PLL13/LConn4 -- D-GND13/LConn1
  VSI-PLL14/LConn4 -- D-GND14/LConn1
  VSI-PLL15/LConn4 -- D-GND15/LConn1
  VSI-PLL16/LConn4 -- D-GND16/LConn1
  VSI-PLL17/LConn4 -- D-GND17/LConn1
  VSI-PLL18/LConn4 -- D-GND18/LConn1
  VSI-PLL20/LConn4 -- D-GND20/LConn1
  VSI-PLL21/LConn4 -- D-GND21/LConn1
  VSI-PLL23/LConn4 -- D-GND23/LConn1
  VSI-PLL24/LConn4 -- D-GND24/LConn1
  VSI-PLL25/LConn4 -- D-GND25/LConn1
  VSI-PLL26/LConn4 -- D-GND26/LConn1
  VSI-PLL27/LConn4 -- D-GND27/LConn1
  VSI-PLL28/LConn4 -- D-GND28/LConn1
  VSI-PLL29/LConn4 -- D-GND29/LConn1
  VSI-PLL33/LConn4 -- D-GND33/LConn1
  VSI-PLL36/LConn4 -- D-GND36/LConn1
  VSI-PLL39/LConn4 -- D-GND39/LConn1
  VSI-PLL40/LConn4 -- D-GND40/LConn1
  VSI-PLL41/LConn4 -- D-GND41/LConn1
  VSI-PLL42/LConn4 -- D-GND42/LConn1
  VSI-PLL44/LConn4 -- D-GND44/LConn1
  VSI-PLL45/LConn4 -- D-GND45/LConn1
  VSI-PLL46/LConn4 -- D-GND46/LConn1
  VSI-PLL47/LConn4 -- D-GND47/LConn1
  VSI-PLL48/LConn4 -- D-GND48/LConn1
  VSI-PLL49/LConn4 -- D-GND49/LConn1
  VSI-PLL50/LConn4 -- D-GND50/LConn1
  VSI-PLL51/LConn4 -- D-GND51/LConn1
  VSI-PLL52/LConn4 -- D-GND52/LConn1
  VSI-PLL53/LConn4 -- D-GND53/LConn1
  VSI-PLL55/LConn4 -- D-GND55/LConn1
  VSI-PLL56/LConn4 -- D-GND56/LConn1
  VSI-PLL59/LConn4 -- D-GND59/LConn1
  VSI-PLL60/LConn4 -- D-GND60/LConn1
  VSI-PLL61/LConn4 -- D-GND61/LConn1
  VSI-PLL64/LConn4 -- D-GND64/LConn1
  VSI-PLL67/LConn4 -- D-GND67/LConn1
  VSI-PLL68/LConn4 -- D-GND68/LConn1
  Branch1-18/RConn1 -- Bus18/RConn1 -- Branch18-50/LConn1 -- Branch18-49/LConn1 -- Branch18-42/LConn1
  Branch1-18/RConn2 -- Bus18/RConn2 -- Branch18-50/LConn2 -- Branch18-49/LConn2 -- Branch18-42/LConn2
  Branch1-18/RConn3 -- Bus18/RConn3 -- Branch18-50/LConn3 -- Branch18-49/LConn3 -- Branch18-42/LConn3
  Bus1/RConn1 -- Branch1-18/LConn1
  Bus1/RConn2 -- Branch1-18/LConn2
  Bus1/RConn3 -- Branch1-18/LConn3
  Branch2-58/RConn1 -- Bus58/RConn1 -- Branch58-63/LConn1 -- Branch58-59/LConn1 -- Branch57-58/RConn1
  Branch2-58/RConn2 -- Bus58/RConn2 -- Branch58-63/LConn2 -- Branch58-59/LConn2 -- Branch57-58/RConn2
  Branch2-58/RConn3 -- Bus58/RConn3 -- Branch58-63/LConn3 -- Branch58-59/LConn3 -- Branch57-58/RConn3
  Transformer2-58/RConn1 -- Branch2-58/LConn1
  Transformer2-58/RConn2 -- Branch2-58/LConn2
  Transformer2-58/RConn3 -- Branch2-58/LConn3
  Bus2/RConn1 -- Transformer2-58/LConn1
  Bus2/RConn2 -- Transformer2-58/LConn2
  Bus2/RConn3 -- Transformer2-58/LConn3
  Branch3-62/RConn1 -- Bus62/RConn1 -- Branch62-65/LConn1 -- Branch62-63/LConn1
  Branch3-62/RConn2 -- Bus62/RConn2 -- Branch62-65/LConn2 -- Branch62-63/LConn2
  Branch3-62/RConn3 -- Bus62/RConn3 -- Branch62-65/LConn3 -- Branch62-63/LConn3
  Transformer3-62/RConn1 -- Branch3-62/LConn1
  Transformer3-62/RConn2 -- Branch3-62/LConn2
  Transformer3-62/RConn3 -- Branch3-62/LConn3
  Bus3/RConn1 -- Transformer3-62/LConn1
  Bus3/RConn2 -- Transformer3-62/LConn2
  Bus3/RConn3 -- Transformer3-62/LConn3
  Branch4-19/RConn1 -- Bus19/RConn1 -- Branch19-68/LConn1 -- Transformer19-20/LConn1
  Branch4-19/RConn2 -- Bus19/RConn2 -- Branch19-68/LConn2 -- Transformer19-20/LConn2
  Branch4-19/RConn3 -- Bus19/RConn3 -- Branch19-68/LConn3 -- Transformer19-20/LConn3
  Transformer4-19/RConn1 -- Branch4-19/LConn1
  Transformer4-19/RConn2 -- Branch4-19/LConn2
  Transformer4-19/RConn3 -- Branch4-19/LConn3
  Bus4/RConn1 -- Transformer4-19/LConn1
  Bus4/RConn2 -- Transformer4-19/LConn2
  Bus4/RConn3 -- Transformer4-19/LConn3
  Branch5-20/RConn1 -- Bus20/RConn1 -- Branch19-20/RConn1
  Branch5-20/RConn2 -- Bus20/RConn2 -- Branch19-20/RConn2
  Branch5-20/RConn3 -- Bus20/RConn3 -- Branch19-20/RConn3
  Transformer5-20/RConn1 -- Branch5-20/LConn1
  Transformer5-20/RConn2 -- Branch5-20/LConn2
  Transformer5-20/RConn3 -- Branch5-20/LConn3
  Bus5/RConn1 -- Transformer5-20/LConn1
  Bus5/RConn2 -- Transformer5-20/LConn2
  Bus5/RConn3 -- Transformer5-20/LConn3
  Branch6-22/RConn1 -- Bus22/RConn1 -- Branch22-23/LConn1 -- Branch21-22/RConn1
  Branch6-22/RConn2 -- Bus22/RConn2 -- Branch22-23/LConn2 -- Branch21-22/RConn2
  Branch6-22/RConn3 -- Bus22/RConn3 -- Branch22-23/LConn3 -- Branch21-22/RConn3
  Transformer6-22/RConn1 -- Branch6-22/LConn1
  Transformer6-22/RConn2 -- Branch6-22/LConn2
  Transformer6-22/RConn3 -- Branch6-22/LConn3
  Bus6/RConn1 -- Transformer6-22/LConn1
  Bus6/RConn2 -- Transformer6-22/LConn2
  Bus6/RConn3 -- Transformer6-22/LConn3
  Branch7-23/RConn1 -- Bus23/RConn1 -- Branch23-24/LConn1 -- Branch22-23/RConn1
  Branch7-23/RConn2 -- Bus23/RConn2 -- Branch23-24/LConn2 -- Branch22-23/RConn2
  Branch7-23/RConn3 -- Bus23/RConn3 -- Branch23-24/LConn3 -- Branch22-23/RConn3
  Bus7/RConn1 -- Branch7-23/LConn1
  Bus7/RConn2 -- Branch7-23/LConn2
  Bus7/RConn3 -- Branch7-23/LConn3
  Branch8-25/RConn1 -- Bus25/RConn1 -- Branch25-54/LConn1 -- Branch25-26/LConn1
  Branch8-25/RConn2 -- Bus25/RConn2 -- Branch25-54/LConn2 -- Branch25-26/LConn2
  Branch8-25/RConn3 -- Bus25/RConn3 -- Branch25-54/LConn3 -- Branch25-26/LConn3
  Transformer8-25/RConn1 -- Branch8-25/LConn1
  Transformer8-25/RConn2 -- Branch8-25/LConn2
  Transformer8-25/RConn3 -- Branch8-25/LConn3
  Bus8/RConn1 -- Transformer8-25/LConn1
  Bus8/RConn2 -- Transformer8-25/LConn2
  Bus8/RConn3 -- Transformer8-25/LConn3
  Branch9-29/RConn1 -- Bus29/RConn1 -- Branch28-29/RConn1 -- Branch26-29/RConn1
  Branch9-29/RConn2 -- Bus29/RConn2 -- Branch28-29/RConn2 -- Branch26-29/RConn2
  Branch9-29/RConn3 -- Bus29/RConn3 -- Branch28-29/RConn3 -- Branch26-29/RConn3
  Transformer9-29/RConn1 -- Branch9-29/LConn1
  Transformer9-29/RConn2 -- Branch9-29/LConn2
  Transformer9-29/RConn3 -- Branch9-29/LConn3
  Bus9/RConn1 -- Transformer9-29/LConn1
  Bus9/RConn2 -- Transformer9-29/LConn2
  Bus9/RConn3 -- Transformer9-29/LConn3
  Branch10-31/RConn1 -- Bus31/RConn1 -- Branch31-53/LConn1 -- Branch31-38/LConn1 -- Branch30-31/RConn1
  Branch10-31/RConn2 -- Bus31/RConn2 -- Branch31-53/LConn2 -- Branch31-38/LConn2 -- Branch30-31/RConn2
  Branch10-31/RConn3 -- Bus31/RConn3 -- Branch31-53/LConn3 -- Branch31-38/LConn3 -- Branch30-31/RConn3
  Transformer10-31/RConn1 -- Branch10-31/LConn1
  Transformer10-31/RConn2 -- Branch10-31/LConn2
  Transformer10-31/RConn3 -- Branch10-31/LConn3
  Bus10/RConn1 -- Transformer10-31/LConn1
  Bus10/RConn2 -- Transformer10-31/LConn2
  Bus10/RConn3 -- Transformer10-31/LConn3
  Branch11-32/RConn1 -- Bus32/RConn1 -- Branch32-33/LConn1 -- Branch30-32/RConn1
  Branch11-32/RConn2 -- Bus32/RConn2 -- Branch32-33/LConn2 -- Branch30-32/RConn2
  Branch11-32/RConn3 -- Bus32/RConn3 -- Branch32-33/LConn3 -- Branch30-32/RConn3
  Transformer11-32/RConn1 -- Branch11-32/LConn1
  Transformer11-32/RConn2 -- Branch11-32/LConn2
  Transformer11-32/RConn3 -- Branch11-32/LConn3
  Bus11/RConn1 -- Transformer11-32/LConn1
  Bus11/RConn2 -- Transformer11-32/LConn2
  Bus11/RConn3 -- Transformer11-32/LConn3
  Branch12-36/RConn1 -- Bus36/RConn1 -- Branch36-61/LConn1 -- Branch34-36/RConn1 -- Branch17-36/RConn1
  Branch12-36/RConn2 -- Bus36/RConn2 -- Branch36-61/LConn2 -- Branch34-36/RConn2 -- Branch17-36/RConn2
  Branch12-36/RConn3 -- Bus36/RConn3 -- Branch36-61/LConn3 -- Branch34-36/RConn3 -- Branch17-36/RConn3
  Transformer12-36/RConn1 -- Branch12-36/LConn1
  Transformer12-36/RConn2 -- Branch12-36/LConn2
  Transformer12-36/RConn3 -- Branch12-36/LConn3
  Bus12/RConn1 -- Transformer12-36/LConn1
  Bus12/RConn2 -- Transformer12-36/LConn2
  Bus12/RConn3 -- Transformer12-36/LConn3
  Branch13-17/RConn1 -- Bus17/RConn1 -- Branch17-43/LConn1 -- Branch17-36/LConn1
  Branch13-17/RConn2 -- Bus17/RConn2 -- Branch17-43/LConn2 -- Branch17-36/LConn2
  Branch13-17/RConn3 -- Bus17/RConn3 -- Branch17-43/LConn3 -- Branch17-36/LConn3
  Transformer13-17/RConn1 -- Branch13-17/LConn1
  Transformer13-17/RConn2 -- Branch13-17/LConn2
  Transformer13-17/RConn3 -- Branch13-17/LConn3
  Bus13/RConn1 -- Transformer13-17/LConn1
  Bus13/RConn2 -- Transformer13-17/LConn2
  Bus13/RConn3 -- Transformer13-17/LConn3
  Branch14-41/RConn1 -- Bus41/RConn1 -- Branch41-42/LConn1 -- Branch40-41/RConn1
  Branch14-41/RConn2 -- Bus41/RConn2 -- Branch41-42/LConn2 -- Branch40-41/RConn2
  Branch14-41/RConn3 -- Bus41/RConn3 -- Branch41-42/LConn3 -- Branch40-41/RConn3
  Bus14/RConn1 -- Branch14-41/LConn1
  Bus14/RConn2 -- Branch14-41/LConn2
  Bus14/RConn3 -- Branch14-41/LConn3
  Branch15-42/RConn1 -- Bus42/RConn1 -- Branch41-42/RConn1 -- Branch18-42/RConn1
  Branch15-42/RConn2 -- Bus42/RConn2 -- Branch41-42/RConn2 -- Branch18-42/RConn2
  Branch15-42/RConn3 -- Bus42/RConn3 -- Branch41-42/RConn3 -- Branch18-42/RConn3
  Bus15/RConn1 -- Branch15-42/LConn1
  Bus15/RConn2 -- Branch15-42/LConn2
  Bus15/RConn3 -- Branch15-42/LConn3
  Branch16-54/RConn1 -- Bus54/RConn1 -- Branch54-55/LConn1 -- Branch53-54/RConn1 -- Branch25-54/RConn1
  Branch16-54/RConn2 -- Bus54/RConn2 -- Branch54-55/LConn2 -- Branch53-54/RConn2 -- Branch25-54/RConn2
  Branch16-54/RConn3 -- Bus54/RConn3 -- Branch54-55/LConn3 -- Branch53-54/RConn3 -- Branch25-54/RConn3
  Transformer16-54/RConn1 -- Branch16-54/LConn1
  Transformer16-54/RConn2 -- Branch16-54/LConn2
  Transformer16-54/RConn3 -- Branch16-54/LConn3
  Bus16/RConn1 -- Transformer16-54/LConn1
  Bus16/RConn2 -- Transformer16-54/LConn2
  Bus16/RConn3 -- Transformer16-54/LConn3
  Branch17-43/RConn1 -- Bus43/RConn1 -- Branch43-44/LConn1
  Branch17-43/RConn2 -- Bus43/RConn2 -- Branch43-44/LConn2
  Branch17-43/RConn3 -- Bus43/RConn3 -- Branch43-44/LConn3
  Branch18-49/RConn1 -- Bus49/RConn1 -- Branch46-49/RConn1
  Branch18-49/RConn2 -- Bus49/RConn2 -- Branch46-49/RConn2
  Branch18-49/RConn3 -- Bus49/RConn3 -- Branch46-49/RConn3
  Branch18-50/RConn1 -- Bus50/RConn1 -- Branch50-51/LConn1
  Branch18-50/RConn2 -- Bus50/RConn2 -- Branch50-51/LConn2
  Branch18-50/RConn3 -- Bus50/RConn3 -- Branch50-51/LConn3
  Transformer19-20/RConn1 -- Branch19-20/LConn1
  Transformer19-20/RConn2 -- Branch19-20/LConn2
  Transformer19-20/RConn3 -- Branch19-20/LConn3
  Branch19-68/RConn1 -- Bus68/RConn1 -- Branch67-68/RConn1 -- Branch37-68/RConn1 -- Branch24-68/RConn1 -- Branch21-68/RConn1
  Branch19-68/RConn2 -- Bus68/RConn2 -- Branch67-68/RConn2 -- Branch37-68/RConn2 -- Branch24-68/RConn2 -- Branch21-68/RConn2
  Branch19-68/RConn3 -- Bus68/RConn3 -- Branch67-68/RConn3 -- Branch37-68/RConn3 -- Branch24-68/RConn3 -- Branch21-68/RConn3
  Branch21-22/LConn1 -- Bus21/RConn1 -- Branch21-68/LConn1
  Branch21-22/LConn2 -- Bus21/RConn2 -- Branch21-68/LConn2
  Branch21-22/LConn3 -- Bus21/RConn3 -- Branch21-68/LConn3
  Branch23-24/RConn1 -- Bus24/RConn1 -- Branch24-68/LConn1
  Branch23-24/RConn2 -- Bus24/RConn2 -- Branch24-68/LConn2
  Branch23-24/RConn3 -- Bus24/RConn3 -- Branch24-68/LConn3
  Branch25-26/RConn1 -- Bus26/RConn1 -- Branch26-29/LConn1 -- Branch26-28/LConn1 -- Branch26-27/LConn1
  Branch25-26/RConn2 -- Bus26/RConn2 -- Branch26-29/LConn2 -- Branch26-28/LConn2 -- Branch26-27/LConn2
  Branch25-26/RConn3 -- Bus26/RConn3 -- Branch26-29/LConn3 -- Branch26-28/LConn3 -- Branch26-27/LConn3
  Branch26-27/RConn1 -- Bus27/RConn1 -- Branch27-53/LConn1 -- Branch27-37/LConn1
  Branch26-27/RConn2 -- Bus27/RConn2 -- Branch27-53/LConn2 -- Branch27-37/LConn2
  Branch26-27/RConn3 -- Bus27/RConn3 -- Branch27-53/LConn3 -- Branch27-37/LConn3
  Branch26-28/RConn1 -- Bus28/RConn1 -- Branch28-29/LConn1
  Branch26-28/RConn2 -- Bus28/RConn2 -- Branch28-29/LConn2
  Branch26-28/RConn3 -- Bus28/RConn3 -- Branch28-29/LConn3
  Branch27-37/RConn1 -- Bus37/RConn1 -- Branch37-68/LConn1 -- Branch37-52/LConn1
  Branch27-37/RConn2 -- Bus37/RConn2 -- Branch37-68/LConn2 -- Branch37-52/LConn2
  Branch27-37/RConn3 -- Bus37/RConn3 -- Branch37-68/LConn3 -- Branch37-52/LConn3
  Branch27-53/RConn1 -- Bus53/RConn1 -- Branch53-54/LConn1 -- Branch47-53/RConn1 -- Branch31-53/RConn1 -- Branch30-53/RConn1
  Branch27-53/RConn2 -- Bus53/RConn2 -- Branch53-54/LConn2 -- Branch47-53/RConn2 -- Branch31-53/RConn2 -- Branch30-53/RConn2
  Branch27-53/RConn3 -- Bus53/RConn3 -- Branch53-54/LConn3 -- Branch47-53/RConn3 -- Branch31-53/RConn3 -- Branch30-53/RConn3
  Branch30-31/LConn1 -- Bus30/RConn1 -- Branch30-61/LConn1 -- Branch30-53/LConn1 -- Branch30-32/LConn1
  Branch30-31/LConn2 -- Bus30/RConn2 -- Branch30-61/LConn2 -- Branch30-53/LConn2 -- Branch30-32/LConn2
  Branch30-31/LConn3 -- Bus30/RConn3 -- Branch30-61/LConn3 -- Branch30-53/LConn3 -- Branch30-32/LConn3
  Branch30-61/RConn1 -- Bus61/RConn1 -- Branch60-61/RConn1 -- Branch36-61/RConn1
  Branch30-61/RConn2 -- Bus61/RConn2 -- Branch60-61/RConn2 -- Branch36-61/RConn2
  Branch30-61/RConn3 -- Bus61/RConn3 -- Branch60-61/RConn3 -- Branch36-61/RConn3
  Branch31-38/RConn1 -- Bus38/RConn1 -- Branch38-46/LConn1 -- Branch33-38/RConn1
  Branch31-38/RConn2 -- Bus38/RConn2 -- Branch38-46/LConn2 -- Branch33-38/RConn2
  Branch31-38/RConn3 -- Bus38/RConn3 -- Branch38-46/LConn3 -- Branch33-38/RConn3
  Branch32-33/RConn1 -- Bus33/RConn1 -- Branch33-38/LConn1 -- Branch33-34/LConn1
  Branch32-33/RConn2 -- Bus33/RConn2 -- Branch33-38/LConn2 -- Branch33-34/LConn2
  Branch32-33/RConn3 -- Bus33/RConn3 -- Branch33-38/LConn3 -- Branch33-34/LConn3
  Branch33-34/RConn1 -- Bus34/RConn1 -- Branch34-36/LConn1 -- Transformer34-35/LConn1
  Branch33-34/RConn2 -- Bus34/RConn2 -- Branch34-36/LConn2 -- Transformer34-35/LConn2
  Branch33-34/RConn3 -- Bus34/RConn3 -- Branch34-36/LConn3 -- Transformer34-35/LConn3
  Branch34-35/RConn1 -- Bus35/RConn1 -- Branch35-45/LConn1
  Branch34-35/RConn2 -- Bus35/RConn2 -- Branch35-45/LConn2
  Branch34-35/RConn3 -- Bus35/RConn3 -- Branch35-45/LConn3
  Transformer34-35/RConn1 -- Branch34-35/LConn1
  Transformer34-35/RConn2 -- Branch34-35/LConn2
  Transformer34-35/RConn3 -- Branch34-35/LConn3
  Branch35-45/RConn1 -- Bus45/RConn1 -- Branch45-51/LConn1 -- Branch44-45/RConn1 -- Branch39-45/RConn1
  Branch35-45/RConn2 -- Bus45/RConn2 -- Branch45-51/LConn2 -- Branch44-45/RConn2 -- Branch39-45/RConn2
  Branch35-45/RConn3 -- Bus45/RConn3 -- Branch45-51/LConn3 -- Branch44-45/RConn3 -- Branch39-45/RConn3
  Branch37-52/RConn1 -- Bus52/RConn1 -- Branch52-55/LConn1
  Branch37-52/RConn2 -- Bus52/RConn2 -- Branch52-55/LConn2
  Branch37-52/RConn3 -- Bus52/RConn3 -- Branch52-55/LConn3
  Branch38-46/RConn1 -- Bus46/RConn1 -- Branch46-49/LConn1
  Branch38-46/RConn2 -- Bus46/RConn2 -- Branch46-49/LConn2
  Branch38-46/RConn3 -- Bus46/RConn3 -- Branch46-49/LConn3
  Branch39-44/RConn1 -- Bus44/RConn1 -- Branch44-45/LConn1 -- Branch43-44/RConn1
  Branch39-44/RConn2 -- Bus44/RConn2 -- Branch44-45/LConn2 -- Branch43-44/RConn2
  Branch39-44/RConn3 -- Bus44/RConn3 -- Branch44-45/LConn3 -- Branch43-44/RConn3
  Branch39-44/LConn1 -- Bus39/RConn1 -- Branch39-45/LConn1
  Branch39-44/LConn2 -- Bus39/RConn2 -- Branch39-45/LConn2
  Branch39-44/LConn3 -- Bus39/RConn3 -- Branch39-45/LConn3
  Branch40-41/LConn1 -- Bus40/RConn1 -- Branch40-48/LConn1
  Branch40-41/LConn2 -- Bus40/RConn2 -- Branch40-48/LConn2
  Branch40-41/LConn3 -- Bus40/RConn3 -- Branch40-48/LConn3
  Branch40-48/RConn1 -- Bus48/RConn1 -- Branch47-48/RConn1
  Branch40-48/RConn2 -- Bus48/RConn2 -- Branch47-48/RConn2
  Branch40-48/RConn3 -- Bus48/RConn3 -- Branch47-48/RConn3
  Branch45-51/RConn1 -- Bus51/RConn1 -- Branch50-51/RConn1
  Branch45-51/RConn2 -- Bus51/RConn2 -- Branch50-51/RConn2
  Branch45-51/RConn3 -- Bus51/RConn3 -- Branch50-51/RConn3
  Branch47-48/LConn1 -- Bus47/RConn1 -- Branch47-53/LConn1
  Branch47-48/LConn2 -- Bus47/RConn2 -- Branch47-53/LConn2
  Branch47-48/LConn3 -- Bus47/RConn3 -- Branch47-53/LConn3
  Branch52-55/RConn1 -- Bus55/RConn1 -- Branch55-56/LConn1 -- Branch54-55/RConn1
  Branch52-55/RConn2 -- Bus55/RConn2 -- Branch55-56/LConn2 -- Branch54-55/RConn2
  Branch52-55/RConn3 -- Bus55/RConn3 -- Branch55-56/LConn3 -- Branch54-55/RConn3
  Branch55-56/RConn1 -- Bus56/RConn1 -- Branch56-66/LConn1 -- Branch56-57/LConn1
  Branch55-56/RConn2 -- Bus56/RConn2 -- Branch56-66/LConn2 -- Branch56-57/LConn2
  Branch55-56/RConn3 -- Bus56/RConn3 -- Branch56-66/LConn3 -- Branch56-57/LConn3
  Branch56-57/RConn1 -- Bus57/RConn1 -- Branch57-60/LConn1 -- Branch57-58/LConn1
  Branch56-57/RConn2 -- Bus57/RConn2 -- Branch57-60/LConn2 -- Branch57-58/LConn2
  Branch56-57/RConn3 -- Bus57/RConn3 -- Branch57-60/LConn3 -- Branch57-58/LConn3
  Branch56-66/RConn1 -- Bus66/RConn1 -- Branch66-67/LConn1 -- Branch65-66/RConn1
  Branch56-66/RConn2 -- Bus66/RConn2 -- Branch66-67/LConn2 -- Branch65-66/RConn2
  Branch56-66/RConn3 -- Bus66/RConn3 -- Branch66-67/LConn3 -- Branch65-66/RConn3
  Branch57-60/RConn1 -- Bus60/RConn1 -- Branch60-61/LConn1 -- Branch59-60/RConn1
  Branch57-60/RConn2 -- Bus60/RConn2 -- Branch60-61/LConn2 -- Branch59-60/RConn2
  Branch57-60/RConn3 -- Bus60/RConn3 -- Branch60-61/LConn3 -- Branch59-60/RConn3
  Branch58-59/RConn1 -- Bus59/RConn1 -- Branch59-60/LConn1
  Branch58-59/RConn2 -- Bus59/RConn2 -- Branch59-60/LConn2
  Branch58-59/RConn3 -- Bus59/RConn3 -- Branch59-60/LConn3
  Branch58-63/RConn1 -- Bus63/RConn1 -- Transformer63-64/LConn1 -- Branch62-63/RConn1
  Branch58-63/RConn2 -- Bus63/RConn2 -- Transformer63-64/LConn2 -- Branch62-63/RConn2
  Branch58-63/RConn3 -- Bus63/RConn3 -- Transformer63-64/LConn3 -- Branch62-63/RConn3
  Branch62-65/RConn1 -- Bus65/RConn1 -- Branch65-66/LConn1 -- Branch64-65/RConn1
  Branch62-65/RConn2 -- Bus65/RConn2 -- Branch65-66/LConn2 -- Branch64-65/RConn2
  Branch62-65/RConn3 -- Bus65/RConn3 -- Branch65-66/LConn3 -- Branch64-65/RConn3
  Branch63-64/RConn1 -- Bus64/RConn1 -- Transformer64-65/LConn1
  Branch63-64/RConn2 -- Bus64/RConn2 -- Transformer64-65/LConn2
  Branch63-64/RConn3 -- Bus64/RConn3 -- Transformer64-65/LConn3
  Transformer63-64/RConn1 -- Branch63-64/LConn1
  Transformer63-64/RConn2 -- Branch63-64/LConn2
  Transformer63-64/RConn3 -- Branch63-64/LConn3
  Transformer64-65/RConn1 -- Branch64-65/LConn1
  Transformer64-65/RConn2 -- Branch64-65/LConn2
  Transformer64-65/RConn3 -- Branch64-65/LConn3
  Branch66-67/RConn1 -- Bus67/RConn1 -- Branch67-68/LConn1
  Branch66-67/RConn2 -- Bus67/RConn2 -- Branch67-68/LConn2
  Branch66-67/RConn3 -- Bus67/RConn3 -- Branch67-68/LConn3
  VSI-PLL1/LConn1 -- Bus1/LConn1
  VSI-PLL1/LConn2 -- Bus1/LConn2
  VSI-PLL1/LConn3 -- Bus1/LConn3
  VSI-PLL2/LConn1 -- Bus2/LConn1
  VSI-PLL2/LConn2 -- Bus2/LConn2
  VSI-PLL2/LConn3 -- Bus2/LConn3
  VSI-PLL3/LConn1 -- Bus3/LConn1
  VSI-PLL3/LConn2 -- Bus3/LConn2
  VSI-PLL3/LConn3 -- Bus3/LConn3
  VSI-PLL4/LConn1 -- Bus4/LConn1
  VSI-PLL4/LConn2 -- Bus4/LConn2
  VSI-PLL4/LConn3 -- Bus4/LConn3
  VSI-PLL5/LConn1 -- Bus5/LConn1
  VSI-PLL5/LConn2 -- Bus5/LConn2
  VSI-PLL5/LConn3 -- Bus5/LConn3
  VSI-PLL6/LConn1 -- Bus6/LConn1
  VSI-PLL6/LConn2 -- Bus6/LConn2
  VSI-PLL6/LConn3 -- Bus6/LConn3
  VSI-PLL7/LConn1 -- Bus7/LConn1
  VSI-PLL7/LConn2 -- Bus7/LConn2
  VSI-PLL7/LConn3 -- Bus7/LConn3
  VSI-PLL8/LConn1 -- Bus8/LConn1
  VSI-PLL8/LConn2 -- Bus8/LConn2
  VSI-PLL8/LConn3 -- Bus8/LConn3
  VSI-PLL9/LConn1 -- Bus9/LConn1
  VSI-PLL9/LConn2 -- Bus9/LConn2
  VSI-PLL9/LConn3 -- Bus9/LConn3
  VSI-PLL10/LConn1 -- Bus10/LConn1
  VSI-PLL10/LConn2 -- Bus10/LConn2
  VSI-PLL10/LConn3 -- Bus10/LConn3
  VSI-PLL11/LConn1 -- Bus11/LConn1
  VSI-PLL11/LConn2 -- Bus11/LConn2
  VSI-PLL11/LConn3 -- Bus11/LConn3
  VSI-PLL12/LConn1 -- Bus12/LConn1
  VSI-PLL12/LConn2 -- Bus12/LConn2
  VSI-PLL12/LConn3 -- Bus12/LConn3
  VSI-PLL13/LConn1 -- Bus13/LConn1
  VSI-PLL13/LConn2 -- Bus13/LConn2
  VSI-PLL13/LConn3 -- Bus13/LConn3
  VSI-PLL14/LConn1 -- Bus14/LConn1
  VSI-PLL14/LConn2 -- Bus14/LConn2
  VSI-PLL14/LConn3 -- Bus14/LConn3
  VSI-PLL15/LConn1 -- Bus15/LConn1
  VSI-PLL15/LConn2 -- Bus15/LConn2
  VSI-PLL15/LConn3 -- Bus15/LConn3
  VSI-PLL16/LConn1 -- Bus16/LConn1
  VSI-PLL16/LConn2 -- Bus16/LConn2
  VSI-PLL16/LConn3 -- Bus16/LConn3
  VSI-PLL17/LConn1 -- Bus17/LConn1
  VSI-PLL17/LConn2 -- Bus17/LConn2
  VSI-PLL17/LConn3 -- Bus17/LConn3
  VSI-PLL18/LConn1 -- Bus18/LConn1
  VSI-PLL18/LConn2 -- Bus18/LConn2
  VSI-PLL18/LConn3 -- Bus18/LConn3
  VSI-PLL20/LConn1 -- Bus20/LConn1
  VSI-PLL20/LConn2 -- Bus20/LConn2
  VSI-PLL20/LConn3 -- Bus20/LConn3
  VSI-PLL21/LConn1 -- Bus21/LConn1
  VSI-PLL21/LConn2 -- Bus21/LConn2
  VSI-PLL21/LConn3 -- Bus21/LConn3
  VSI-PLL23/LConn1 -- Bus23/LConn1
  VSI-PLL23/LConn2 -- Bus23/LConn2
  VSI-PLL23/LConn3 -- Bus23/LConn3
  VSI-PLL24/LConn1 -- Bus24/LConn1
  VSI-PLL24/LConn2 -- Bus24/LConn2
  VSI-PLL24/LConn3 -- Bus24/LConn3
  VSI-PLL25/LConn1 -- Bus25/LConn1
  VSI-PLL25/LConn2 -- Bus25/LConn2
  VSI-PLL25/LConn3 -- Bus25/LConn3
  VSI-PLL26/LConn1 -- Bus26/LConn1
  VSI-PLL26/LConn2 -- Bus26/LConn2
  VSI-PLL26/LConn3 -- Bus26/LConn3
  VSI-PLL27/LConn1 -- Bus27/LConn1
  VSI-PLL27/LConn2 -- Bus27/LConn2
  VSI-PLL27/LConn3 -- Bus27/LConn3
  VSI-PLL28/LConn1 -- Bus28/LConn1
  VSI-PLL28/LConn2 -- Bus28/LConn2
  VSI-PLL28/LConn3 -- Bus28/LConn3
  VSI-PLL29/LConn1 -- Bus29/LConn1
  VSI-PLL29/LConn2 -- Bus29/LConn2
  VSI-PLL29/LConn3 -- Bus29/LConn3
  VSI-PLL33/LConn1 -- Bus33/LConn1
  VSI-PLL33/LConn2 -- Bus33/LConn2
  VSI-PLL33/LConn3 -- Bus33/LConn3
  VSI-PLL36/LConn1 -- Bus36/LConn1
  VSI-PLL36/LConn2 -- Bus36/LConn2
  VSI-PLL36/LConn3 -- Bus36/LConn3
  VSI-PLL39/LConn1 -- Bus39/LConn1
  VSI-PLL39/LConn2 -- Bus39/LConn2
  VSI-PLL39/LConn3 -- Bus39/LConn3
  VSI-PLL40/LConn1 -- Bus40/LConn1
  VSI-PLL40/LConn2 -- Bus40/LConn2
  VSI-PLL40/LConn3 -- Bus40/LConn3
  VSI-PLL41/LConn1 -- Bus41/LConn1
  VSI-PLL41/LConn2 -- Bus41/LConn2
  VSI-PLL41/LConn3 -- Bus41/LConn3
  VSI-PLL42/LConn1 -- Bus42/LConn1
  VSI-PLL42/LConn2 -- Bus42/LConn2
  VSI-PLL42/LConn3 -- Bus42/LConn3
  VSI-PLL44/LConn1 -- Bus44/LConn1
  VSI-PLL44/LConn2 -- Bus44/LConn2
  VSI-PLL44/LConn3 -- Bus44/LConn3
  VSI-PLL45/LConn1 -- Bus45/LConn1
  VSI-PLL45/LConn2 -- Bus45/LConn2
  VSI-PLL45/LConn3 -- Bus45/LConn3
  VSI-PLL46/LConn1 -- Bus46/LConn1
  VSI-PLL46/LConn2 -- Bus46/LConn2
  VSI-PLL46/LConn3 -- Bus46/LConn3
  VSI-PLL47/LConn1 -- Bus47/LConn1
  VSI-PLL47/LConn2 -- Bus47/LConn2
  VSI-PLL47/LConn3 -- Bus47/LConn3
  VSI-PLL48/LConn1 -- Bus48/LConn1
  VSI-PLL48/LConn2 -- Bus48/LConn2
  VSI-PLL48/LConn3 -- Bus48/LConn3
  VSI-PLL49/LConn1 -- Bus49/LConn1
  VSI-PLL49/LConn2 -- Bus49/LConn2
  VSI-PLL49/LConn3 -- Bus49/LConn3
  VSI-PLL50/LConn1 -- Bus50/LConn1
  VSI-PLL50/LConn2 -- Bus50/LConn2
  VSI-PLL50/LConn3 -- Bus50/LConn3
  VSI-PLL51/LConn1 -- Bus51/LConn1
  VSI-PLL51/LConn2 -- Bus51/LConn2
  VSI-PLL51/LConn3 -- Bus51/LConn3
  VSI-PLL52/LConn1 -- Bus52/LConn1
  VSI-PLL52/LConn2 -- Bus52/LConn2
  VSI-PLL52/LConn3 -- Bus52/LConn3
  VSI-PLL53/LConn1 -- Bus53/LConn1
  VSI-PLL53/LConn2 -- Bus53/LConn2
  VSI-PLL53/LConn3 -- Bus53/LConn3
  VSI-PLL55/LConn1 -- Bus55/LConn1
  VSI-PLL55/LConn2 -- Bus55/LConn2
  VSI-PLL55/LConn3 -- Bus55/LConn3
  VSI-PLL56/LConn1 -- Bus56/LConn1
  VSI-PLL56/LConn2 -- Bus56/LConn2
  VSI-PLL56/LConn3 -- Bus56/LConn3
  VSI-PLL59/LConn1 -- Bus59/LConn1
  VSI-PLL59/LConn2 -- Bus59/LConn2
  VSI-PLL59/LConn3 -- Bus59/LConn3
  VSI-PLL60/LConn1 -- Bus60/LConn1
  VSI-PLL60/LConn2 -- Bus60/LConn2
  VSI-PLL60/LConn3 -- Bus60/LConn3
  VSI-PLL61/LConn1 -- Bus61/LConn1
  VSI-PLL61/LConn2 -- Bus61/LConn2
  VSI-PLL61/LConn3 -- Bus61/LConn3
  VSI-PLL64/LConn1 -- Bus64/LConn1
  VSI-PLL64/LConn2 -- Bus64/LConn2
  VSI-PLL64/LConn3 -- Bus64/LConn3
  VSI-PLL67/LConn1 -- Bus67/LConn1
  VSI-PLL67/LConn2 -- Bus67/LConn2
  VSI-PLL67/LConn3 -- Bus67/LConn3
  VSI-PLL68/LConn1 -- Bus68/LConn1
  VSI-PLL68/LConn2 -- Bus68/LConn2
  VSI-PLL68/LConn3 -- Bus68/LConn3
  Bus37/LConn3 -- Current Measurement1/LConn1
  Load Impulse1/LConn3 -- Current Measurement1/RConn1
  Bus37/LConn1 -- Load Impulse1/LConn1
  D-GND22/LConn1 -- Load Impulse1/RConn1
  Bus37/LConn2 -- Load Impulse1/LConn2
